simulink model "kinovaMicoSimscapeModel"  (R2021b)
(part 28 of 50)

Y4_10_2=(111*dq5*dqr3*sin(q4))/4000 - (111*dq5*dqr2*sin(q4))/4000 - dq5*dqr4*sin(q5)*((111*3^(1/2))/8000 + 1923/80000) + (111*dq5*dqr2*cos(2*q5)*sin(q4))/4000 + (111*dq5*dqr2*sin(2*q5)*cos(q4))/8000 - (111*dq5*dqr3*cos(2*q5)*sin(q4))/4000 - (111*dq5*dqr3*sin(2*q5)*cos(q4))/8000 + dq2*dqr2*sin(2*q4)*((37*3^(1/2))/16000 + 1923/80000) - dq2*dqr3*sin(2*q4)*((37*3^(1/2))/16000 + 1923/80000) - dq3*dqr2*sin(2*q4)*((37*3^(1/2))/16000 + 1923/80000) + dq3*dqr3*sin(2*q4)*((37*3^(1/2))/16000 + 1923/80000) - dq1*dqr1*sin(2*q4)*((37*3^(1/2))/32000 + 1923/160000) - (111*3^(1/2)*dq5*dqr4*sin(2*q5))/8000 - (29*3^(1/2)*dq1*dqr2*cos(q2)*sin(q4))/400 + (29*3^(1/2)*dq2*dqr2*cos(q4)*sin(q3))/400 - dq2*dqr2*cos(2*q4)*sin(q5)*((111*3^(1/2))/4000 + 1923/40000) + dq2*dqr3*cos(2*q4)*sin(q5)*((111*3^(1/2))/4000 + 1923/40000) + dq3*dqr2*cos(2*q4)*sin(q5)*((111*3^(1/2))/4000 + 1923/40000) - dq3*dqr3*cos(2*q4)*sin(q5)*((111*3^(1/2))/4000 + 1923/40000) - dq2*dqr2*sin(2*q4)*cos(q5)*((111*3^(1/2))/8000 + 1923/80000) + dq2*dqr3*sin(2*q4)*cos(q5)*((111*3^(1/2))/8000 + 1923/80000) + dq3*dqr2*sin(2*q4)*cos(q5)*((111*3^(1/2))/8000 + 1923/80000) - dq3*dqr3*sin(2*q4)*cos(q5)*((111*3^(1/2))/8000 + 1923/80000) + (111*dq1*dqr5*cos(q3)*cos(q4)*sin(q2))/4000 - (37*3^(1/2)*dq1*dqr1*cos(2*q4)*sin(2*q5))/8000 - (37*3^(1/2)*dq1*dqr1*cos(2*q5)*sin(2*q4))/6400 + (37*3^(1/2)*dq2*dqr2*cos(2*q4)*sin(2*q5))/4000 + (37*3^(1/2)*dq2*dqr2*cos(2*q5)*sin(2*q4))/3200 - (37*3^(1/2)*dq2*dqr3*cos(2*q4)*sin(2*q5))/4000 - (37*3^(1/2)*dq2*dqr3*cos(2*q5)*sin(2*q4))/3200 - (37*3^(1/2)*dq3*dqr2*cos(2*q4)*sin(2*q5))/4000 - (37*3^(1/2)*dq3*dqr2*cos(2*q5)*sin(2*q4))/3200 + (37*3^(1/2)*dq3*dqr3*cos(2*q4)*sin(2*q5))/4000 + (37*3^(1/2)*dq3*dqr3*cos(2*q5)*sin(2*q4))/3200 - dq5*dqr2*cos(q4)*sin(q5)*((1923*3^(1/2))/80000 + 333/8000) + dq5*dqr3*cos(q4)*sin(q5)*((1923*3^(1/2))/80000 + 333/8000) - dq1*dqr2*cos(q2)*sin(q3)*((333*3^(1/2))/16000 + 1923/80000) + dq1*dqr2*cos(q3)*sin(q2)*((333*3^(1/2))/16000 + 1923/80000) + dq1*dqr3*cos(q2)*sin(q3)*((333*3^(1/2))/16000 + 1923/80000) - dq1*dqr3*cos(q3)*sin(q2)*((333*3^(1/2))/16000 + 1923/80000) - (111*dq1*dqr2*cos(2*q5)*sin(q2)*sin(q3)*sin(q4))/8000 - (111*dq1*dqr2*sin(2*q5)*cos(q4)*sin(q2)*sin(q3))/4000 + (111*dq1*dqr3*cos(2*q5)*sin(q2)*sin(q3)*sin(q4))/8000 + (111*dq1*dqr3*sin(2*q5)*cos(q4)*sin(q2)*sin(q3))/4000 - (111*dq1*dqr5*sin(2*q5)*cos(q2)*sin(q3)*sin(q4))/8000 + (111*dq1*dqr5*sin(2*q5)*cos(q3)*sin(q2)*sin(q4))/8000 + (29*3^(1/2)*dq1*dqr2*cos(q2)*cos(q4)*sin(q5))/200 + (29*3^(1/2)*dq1*dqr2*cos(q2)*cos(q5)*sin(q4))/400 - (29*3^(1/2)*dq2*dqr2*cos(q4)*cos(q5)*sin(q3))/400 + dq1*dqr2*cos(2*q4)*cos(q2)*sin(q3)*((37*3^(1/2))/16000 + 1923/80000) - dq1*dqr2*cos(2*q4)*cos(q3)*sin(q2)*((37*3^(1/2))/16000 + 1923/80000) - dq1*dqr3*cos(2*q4)*cos(q2)*sin(q3)*((37*3^(1/2))/16000 + 1923/80000) + dq1*dqr3*cos(2*q4)*cos(q3)*sin(q2)*((37*3^(1/2))/16000 + 1923/80000) + (29*3^(1/2)*dq2*dqr2*sin(q3)*sin(q4)*sin(q5))/200 + (111*3^(1/2)*dq1*dqr2*cos(2*q5)*cos(q2)*sin(q3))/16000 - (111*3^(1/2)*dq1*dqr2*cos(2*q5)*cos(q3)*sin(q2))/16000 - (111*3^(1/2)*dq1*dqr3*cos(2*q5)*cos(q2)*sin(q3))/16000 + (111*3^(1/2)*dq1*dqr3*cos(2*q5)*cos(q3)*sin(q2))/16000 - (111*3^(1/2)*dq1*dqr5*sin(2*q5)*sin(q2)*sin(q3))/8000 + dq1*dqr2*cos(q2)*cos(q3)*sin(q4)*((2513*3^(1/2))/40000 - 37/8000) - dq1*dqr3*cos(q2)*cos(q3)*sin(q4)*((2513*3^(1/2))/40000 - 37/8000) + dq1*dqr2*cos(q2)*cos(q5)*sin(q3)*((111*3^(1/2))/8000 + 1923/80000) - dq1*dqr2*cos(q3)*cos(q5)*sin(q2)*((111*3^(1/2))/8000 + 1923/80000) - dq1*dqr3*cos(q2)*cos(q5)*sin(q3)*((111*3^(1/2))/8000 + 1923/80000) + dq1*dqr3*cos(q3)*cos(q5)*sin(q2)*((111*3^(1/2))/8000 + 1923/80000) - (111*dq1*dqr2*cos(2*q5)*cos(q2)*cos(q3)*sin(q4))/8000 - (111*dq1*dqr2*sin(2*q5)*cos(q2)*cos(q3)*cos(q4))/4000 + (111*dq1*dqr3*cos(2*q5)*cos(q2)*cos(q3)*sin(q4))/8000 + (111*dq1*dqr3*sin(2*q5)*cos(q2)*cos(q3)*cos(q4))/4000 - (111*dq1*dqr5*cos(2*q5)*cos(q3)*cos(q4)*sin(q2))/4000 + dq1*dqr2*sin(q2)*sin(q3)*sin(q4)*((2513*3^(1/2))/40000 - 37/8000) - dq1*dqr3*sin(q2)*sin(q3)*sin(q4)*((2513*3^(1/2))/40000 - 37/8000) - dq1*dqr5*sin(q2)*sin(q3)*sin(q5)*((111*3^(1/2))/8000 + 1923/80000) - dq1*dqr2*cos(2*q4)*cos(q2)*cos(q5)*sin(q3)*((111*3^(1/2))/8000 + 1923/80000) + dq1*dqr2*cos(2*q4)*cos(q3)*cos(q5)*sin(q2)*((111*3^(1/2))/8000 + 1923/80000) + dq1*dqr3*cos(2*q4)*cos(q2)*cos(q5)*sin(q3)*((111*3^(1/2))/8000 + 1923/80000) - dq1*dqr3*cos(2*q4)*cos(q3)*cos(q5)*sin(q2)*((111*3^(1/2))/8000 + 1923/80000) + dq1*dqr2*sin(2*q4)*cos(q2)*sin(q3)*sin(q5)*((111*3^(1/2))/4000 + 1923/40000) - dq1*dqr2*sin(2*q4)*cos(q3)*sin(q2)*sin(q5)*((111*3^(1/2))/4000 + 1923/40000) - dq1*dqr3*sin(2*q4)*cos(q2)*sin(q3)*sin(q5)*((111*3^(1/2))/4000 + 1923/40000) + dq1*dqr3*sin(2*q4)*cos(q3)*sin(q2)*sin(q5)*((111*3^(1/2))/4000 + 1923/40000) + (37*3^(1/2)*dq1*dqr1*cos(2*q2)*cos(2*q3)*cos(2*q4)*sin(2*q5))/8000 + (37*3^(1/2)*dq1*dqr2*cos(2*q4)*cos(2*q5)*cos(q2)*sin(q3))/3200 - (37*3^(1/2)*dq1*dqr2*cos(2*q4)*cos(2*q5)*cos(q3)*sin(q2))/3200 - (37*3^(1/2)*dq1*dqr3*cos(2*q4)*cos(2*q5)*cos(q2)*sin(q3))/3200 + (37*3^(1/2)*dq1*dqr3*cos(2*q4)*cos(2*q5)*cos(q3)*sin(q2))/3200 - dq1*dqr2*cos(q2)*cos(q3)*cos(q4)*sin(q5)*((877*3^(1/2))/8000 + 37/4000) + dq1*dqr3*cos(q2)*cos(q3)*cos(q4)*sin(q5)*((877*3^(1/2))/8000 + 37/4000) - dq1*dqr2*cos(q2)*cos(q3)*cos(q5)*sin(q4)*((1231*3^(1/2))/40000 - 37/1000) + dq1*dqr3*cos(q2)*cos(q3)*cos(q5)*sin(q4)*((1231*3^(1/2))/40000 - 37/1000) - (37*3^(1/2)*dq1*dqr2*sin(2*q4)*sin(2*q5)*cos(q2)*sin(q3))/4000 + (37*3^(1/2)*dq1*dqr2*sin(2*q4)*sin(2*q5)*cos(q3)*sin(q2))/4000 + (37*3^(1/2)*dq1*dqr3*sin(2*q4)*sin(2*q5)*cos(q2)*sin(q3))/4000 - (37*3^(1/2)*dq1*dqr3*sin(2*q4)*sin(2*q5)*cos(q3)*sin(q2))/4000 - dq1*dqr2*cos(q4)*sin(q2)*sin(q3)*sin(q5)*((877*3^(1/2))/8000 + 37/4000) + dq1*dqr3*cos(q4)*sin(q2)*sin(q3)*sin(q5)*((877*3^(1/2))/8000 + 37/4000) - dq1*dqr2*cos(q5)*sin(q2)*sin(q3)*sin(q4)*((1231*3^(1/2))/40000 - 37/1000) + dq1*dqr3*cos(q5)*sin(q2)*sin(q3)*sin(q4)*((1231*3^(1/2))/40000 - 37/1000) + dq1*dqr5*cos(q2)*sin(q3)*sin(q4)*sin(q5)*((1923*3^(1/2))/80000 + 333/8000) - dq1*dqr5*cos(q3)*sin(q2)*sin(q4)*sin(q5)*((1923*3^(1/2))/80000 + 333/8000);
Y4_10_3=(333*ddqr1*cos(q2 - q3 + q4 + 2*q5))/32000 - (111*ddqr1*cos(q2 - q3 + q4 - 2*q5))/32000 - (333*ddqr1*cos(q3 - q2 + q4 + 2*q5))/32000 - (37*3^(1/2)*ddqr5)/2000 + (111*ddqr1*cos(q2 - q3 - q4 + 2*q5))/32000 + (111*ddqr2*cos(q4 - 2*q5))/16000 - (333*ddqr2*cos(q4 + 2*q5))/16000 - (111*ddqr3*cos(q4 - 2*q5))/16000 + (333*ddqr3*cos(q4 + 2*q5))/16000 - ddqr4*((333*3^(1/2))/8000 + 1923/40000) - (111*dq2*dqr5*sin(q4))/4000 + (111*dq3*dqr5*sin(q4))/4000 - (29*3^(1/2)*ddqr1*cos(q2 - q4))/800 - (29*3^(1/2)*ddqr2*cos(q3 - q4))/800 + ddqr1*cos(q2 - q3 - q4 + q5)*((403*3^(1/2))/20000 + 37/3200) - ddqr1*cos(q2 - q3 + q4 - q5)*((771*3^(1/2))/40000 + 37/3200) - (87*3^(1/2)*ddqr1*cos(q2 + q4 + q5))/1600 + (87*3^(1/2)*ddqr2*cos(q3 + q4 + q5))/1600 + (111*3^(1/2)*ddqr4*cos(2*q5))/8000 + ddqr1*cos(q2 - q3 + q5)*((111*3^(1/2))/8000 + 1923/80000) + ddqr1*cos(q3 - q2 + q5)*((111*3^(1/2))/8000 + 1923/80000) - ddqr1*cos(q2 - q3 + q4)*((2443*3^(1/2))/80000 - 37/16000) + ddqr1*cos(q3 - q2 + q4)*((2583*3^(1/2))/80000 - 37/16000) - ddqr2*cos(q4 + q5)*((351*3^(1/2))/5000 - 111/8000) + ddqr3*cos(q4 + q5)*((351*3^(1/2))/5000 - 111/8000) + (29*3^(1/2)*ddqr1*cos(q2 + q4 - q5))/1600 - (29*3^(1/2)*ddqr1*cos(q2 - q4 + q5))/1600 + (87*3^(1/2)*ddqr1*cos(q4 - q2 + q5))/1600 - (29*3^(1/2)*ddqr2*cos(q3 + q4 - q5))/1600 - (29*3^(1/2)*ddqr2*cos(q3 - q4 + q5))/1600 + (87*3^(1/2)*ddqr2*cos(q4 - q3 + q5))/1600 + ddqr4*cos(q5)*((111*3^(1/2))/4000 + 1923/40000) + ddqr5*cos(q5)*((111*3^(1/2))/4000 + 1923/40000) + ddqr2*cos(q4)*((2513*3^(1/2))/40000 - 37/8000) - ddqr3*cos(q4)*((2513*3^(1/2))/40000 - 37/8000) + (29*3^(1/2)*ddqr1*cos(q2 + q4))/800 - (29*3^(1/2)*ddqr2*cos(q3 + q4))/800 + ddqr1*cos(q2 - q3 + q4 + q5)*((2703*3^(1/2))/80000 - 111/16000) - ddqr1*cos(q3 - q2 + q4 + q5)*((2913*3^(1/2))/80000 - 111/16000) + ddqr2*cos(q4 - q5)*((1577*3^(1/2))/40000 + 37/1600) - ddqr3*cos(q4 - q5)*((1577*3^(1/2))/40000 + 37/1600) - ddqr1*cos(q2 - q3)*((333*3^(1/2))/8000 + 1923/40000) + (111*3^(1/2)*ddqr1*cos(q2 - q3 + 2*q5))/16000 + (111*3^(1/2)*ddqr1*cos(q3 - q2 + 2*q5))/16000 - dq5*dqr5*sin(q5)*((111*3^(1/2))/4000 + 1923/40000) - dq4*dqr5*sin(q5)*((111*3^(1/2))/8000 + 1923/80000) + (111*dq2*dqr5*cos(2*q5)*sin(q4))/4000 + (111*dq2*dqr5*sin(2*q5)*cos(q4))/8000 - (111*dq3*dqr5*cos(2*q5)*sin(q4))/4000 - (111*dq3*dqr5*sin(2*q5)*cos(q4))/8000 - (111*3^(1/2)*dq4*dqr5*sin(2*q5))/8000 - (111*dq1*dqr5*cos(q2)*cos(q4)*sin(q3))/4000 - dq2*dqr5*cos(q4)*sin(q5)*((1923*3^(1/2))/80000 + 333/8000) + dq3*dqr5*cos(q4)*sin(q5)*((1923*3^(1/2))/80000 + 333/8000) - (111*3^(1/2)*dq1*dqr5*sin(2*q5)*cos(q2)*cos(q3))/8000 - dq1*dqr5*cos(q2)*cos(q3)*sin(q5)*((111*3^(1/2))/8000 + 1923/80000) + (111*dq1*dqr5*cos(2*q5)*cos(q2)*cos(q4)*sin(q3))/4000;
Y4_13_1=(37*sin(q2 - q3)*cos(q4))/1000;
Y4_14_1=(37*cos(q4 - q5)*sin(q2 - q3))/4000 - (111*sin(q2 - q3)*cos(q4 + q5))/4000 + sin(q2 - q3)*cos(q4)*((641*3^(1/2))/20000 + 37/1000);
Y4_18_1=(3*ddqr4)/4 + (3*ddqr1*cos(q2 - q3))/4 + (3*dq1*dqr1*sin(2*q4))/16 - (3*dq2*dqr2*sin(2*q4))/8 + (3*dq2*dqr3*sin(2*q4))/8 + (3*dq3*dqr2*sin(2*q4))/8 - (3*dq3*dqr3*sin(2*q4))/8 + (3^(1/2)*ddqr1*cos(q2 - q3 + q4))/8 - (3^(1/2)*ddqr1*cos(q3 - q2 + q4))/8 - (3^(1/2)*ddqr2*cos(q4))/4 + (3^(1/2)*ddqr3*cos(q4))/4 + (3*dq1*dqr2*cos(q2)*sin(q3))/8 - (3*dq1*dqr2*cos(q3)*sin(q2))/8 + (3*dq2*dqr1*cos(q2)*sin(q3))/8 - (3*dq2*dqr1*cos(q3)*sin(q2))/8 - (3*dq1*dqr3*cos(q2)*sin(q3))/8 + (3*dq1*dqr3*cos(q3)*sin(q2))/8 - (3*dq3*dqr1*cos(q2)*sin(q3))/8 + (3*dq3*dqr1*cos(q3)*sin(q2))/8 - (3*dq1*dqr2*cos(2*q4)*cos(q2)*sin(q3))/8 + (3*dq1*dqr2*cos(2*q4)*cos(q3)*sin(q2))/8 - (3*dq2*dqr1*cos(2*q4)*cos(q2)*sin(q3))/8 + (3*dq2*dqr1*cos(2*q4)*cos(q3)*sin(q2))/8 + (3*dq1*dqr3*cos(2*q4)*cos(q2)*sin(q3))/8 - (3*dq1*dqr3*cos(2*q4)*cos(q3)*sin(q2))/8 + (3*dq3*dqr1*cos(2*q4)*cos(q2)*sin(q3))/8 - (3*dq3*dqr1*cos(2*q4)*cos(q3)*sin(q2))/8 - (3*dq1*dqr1*cos(2*q2)*cos(2*q3)*sin(2*q4))/16 - (3*dq1*dqr1*sin(2*q2)*sin(2*q3)*sin(2*q4))/16 - (3^(1/2)*dq1*dqr2*cos(q2)*cos(q3)*sin(q4))/4 - (3^(1/2)*dq2*dqr1*cos(q2)*cos(q3)*sin(q4))/4 + (3^(1/2)*dq1*dqr3*cos(q2)*cos(q3)*sin(q4))/4 + (3^(1/2)*dq3*dqr1*cos(q2)*cos(q3)*sin(q4))/4 - (3^(1/2)*dq1*dqr2*sin(q2)*sin(q3)*sin(q4))/4 - (3^(1/2)*dq2*dqr1*sin(q2)*sin(q3)*sin(q4))/4 + (3^(1/2)*dq1*dqr3*sin(q2)*sin(q3)*sin(q4))/4 + (3^(1/2)*dq3*dqr1*sin(q2)*sin(q3)*sin(q4))/4 - (3^(1/2)*dq1*dqr1*cos(2*q2)*sin(2*q3)*cos(q4))/8 + (3^(1/2)*dq1*dqr1*cos(2*q3)*sin(2*q2)*cos(q4))/8;
Y4_19_1=(3*dq1*dqr1*cos(2*q4)*sin(2*q5))/32 - (3*dq1*dqr1*cos(2*q4)*sin(q5))/16 - (3*dq1*dqr1*sin(2*q4)*cos(q5))/32 - (3*dq1*dqr1*sin(2*q4))/128 + (15*dq1*dqr1*cos(2*q5)*sin(2*q4))/128 + (21*dq2*dqr1*cos(q2)*sin(q3))/64 - (21*dq2*dqr1*cos(q3)*sin(q2))/64 - (21*dq3*dqr1*cos(q2)*sin(q3))/64 + (21*dq3*dqr1*cos(q3)*sin(q2))/64 - (3*dq1*dqr2*cos(2*q4)*cos(q3)*sin(q2))/64 + (3*dq2*dqr1*cos(2*q4)*cos(q2)*sin(q3))/64 - (3*dq2*dqr1*cos(2*q4)*cos(q3)*sin(q2))/64 - (9*dq2*dqr1*cos(2*q5)*cos(q2)*sin(q3))/64 + (9*dq2*dqr1*cos(2*q5)*cos(q3)*sin(q2))/64 - (3*dq3*dqr1*cos(2*q4)*cos(q2)*sin(q3))/64 + (3*dq3*dqr1*cos(2*q4)*cos(q3)*sin(q2))/64 + (9*dq3*dqr1*cos(2*q5)*cos(q2)*sin(q3))/64 - (9*dq3*dqr1*cos(2*q5)*cos(q3)*sin(q2))/64 + (9*dq5*dqr1*sin(2*q5)*cos(q2)*cos(q3))/32 + (9*dq5*dqr1*sin(2*q5)*sin(q2)*sin(q3))/32 + (3*dq1*dqr2*cos(q3)*cos(q5)*sin(q2))/16 - (3*dq2*dqr1*cos(q2)*cos(q5)*sin(q3))/16 + (3*dq2*dqr1*cos(q3)*cos(q5)*sin(q2))/16 + (3*dq3*dqr1*cos(q2)*cos(q5)*sin(q3))/16 - (3*dq3*dqr1*cos(q3)*cos(q5)*sin(q2))/16 + (3*dq5*dqr1*cos(q2)*cos(q3)*sin(q5))/16 + (3*dq1*dqr1*cos(2*q2)*cos(2*q3)*sin(2*q4))/128 + (3*dq5*dqr1*sin(q2)*sin(q3)*sin(q5))/16 + (3*dq1*dqr1*sin(2*q2)*sin(2*q3)*sin(2*q4))/128 - (3*dq1*dqr1*cos(2*q2)*cos(2*q3)*cos(2*q4)*sin(2*q5))/32 - (15*dq1*dqr1*cos(2*q2)*cos(2*q3)*cos(2*q5)*sin(2*q4))/128 + (3*dq1*dqr2*sin(2*q4)*cos(q3)*sin(q2)*sin(q5))/8 - (3*dq2*dqr1*sin(2*q4)*cos(q2)*sin(q3)*sin(q5))/8 + (3*dq2*dqr1*sin(2*q4)*cos(q3)*sin(q2)*sin(q5))/8 + (3*dq3*dqr1*sin(2*q4)*cos(q2)*sin(q3)*sin(q5))/8 - (3*dq3*dqr1*sin(2*q4)*cos(q3)*sin(q2)*sin(q5))/8 + (3^(1/2)*dq2*dqr1*cos(q2)*cos(q3)*sin(q4))/32 - (3^(1/2)*dq3*dqr1*cos(q2)*cos(q3)*sin(q4))/32 + (3*3^(1/2)*dq5*dqr1*cos(q2)*cos(q4)*sin(q3))/16 - (3*3^(1/2)*dq5*dqr1*cos(q3)*cos(q4)*sin(q2))/16 - (3*dq1*dqr1*cos(2*q4)*sin(2*q2)*sin(2*q3)*sin(2*q5))/32 - (15*dq1*dqr1*cos(2*q5)*sin(2*q2)*sin(2*q3)*sin(2*q4))/128 + (3^(1/2)*dq1*dqr2*sin(q2)*sin(q3)*sin(q4))/32 + (3^(1/2)*dq2*dqr1*sin(q2)*sin(q3)*sin(q4))/32 - (3^(1/2)*dq3*dqr1*sin(q2)*sin(q3)*sin(q4))/32 + (15*dq1*dqr2*cos(2*q4)*cos(2*q5)*cos(q3)*sin(q2))/64 - (15*dq2*dqr1*cos(2*q4)*cos(2*q5)*cos(q2)*sin(q3))/64 + (15*dq2*dqr1*cos(2*q4)*cos(2*q5)*cos(q3)*sin(q2))/64 + (15*dq3*dqr1*cos(2*q4)*cos(2*q5)*cos(q2)*sin(q3))/64 - (15*dq3*dqr1*cos(2*q4)*cos(2*q5)*cos(q3)*sin(q2))/64 - (3*dq1*dqr2*sin(2*q4)*sin(2*q5)*cos(q3)*sin(q2))/16 + (3*dq2*dqr1*sin(2*q4)*sin(2*q5)*cos(q2)*sin(q3))/16 - (3*dq2*dqr1*sin(2*q4)*sin(2*q5)*cos(q3)*sin(q2))/16 - (3*dq3*dqr1*sin(2*q4)*sin(2*q5)*cos(q2)*sin(q3))/16 + (3*dq3*dqr1*sin(2*q4)*sin(2*q5)*cos(q3)*sin(q2))/16 + (3*dq1*dqr1*cos(2*q2)*cos(2*q3)*cos(2*q4)*sin(q5))/16 + (3*dq1*dqr1*cos(2*q2)*cos(2*q3)*sin(2*q4)*cos(q5))/32 + (3*dq1*dqr1*cos(2*q4)*sin(2*q2)*sin(2*q3)*sin(q5))/16 + (3*dq1*dqr1*sin(2*q2)*sin(2*q3)*sin(2*q4)*cos(q5))/32 + (3^(1/2)*dq1*dqr1*cos(2*q2)*sin(2*q3)*cos(q4))/64 - (3^(1/2)*dq1*dqr1*cos(2*q3)*sin(2*q2)*cos(q4))/64 - (3*dq1*dqr2*cos(2*q4)*cos(q3)*cos(q5)*sin(q2))/16 + (3*dq2*dqr1*cos(2*q4)*cos(q2)*cos(q5)*sin(q3))/16 - (3*dq2*dqr1*cos(2*q4)*cos(q3)*cos(q5)*sin(q2))/16 - (3*dq3*dqr1*cos(2*q4)*cos(q2)*cos(q5)*sin(q3))/16 + (3*dq3*dqr1*cos(2*q4)*cos(q3)*cos(q5)*sin(q2))/16 + (3*3^(1/2)*dq1*dqr1*cos(2*q2)*cos(2*q5)*sin(2*q3)*cos(q4))/64 - (3*3^(1/2)*dq1*dqr1*cos(2*q3)*cos(2*q5)*sin(2*q2)*cos(q4))/64 + (3^(1/2)*dq1*dqr2*cos(q4)*sin(q2)*sin(q3)*sin(q5))/8 - (3^(1/2)*dq1*dqr2*cos(q5)*sin(q2)*sin(q3)*sin(q4))/8 + (3^(1/2)*dq2*dqr1*cos(q4)*sin(q2)*sin(q3)*sin(q5))/8 - (3^(1/2)*dq2*dqr1*cos(q5)*sin(q2)*sin(q3)*sin(q4))/8 - (3^(1/2)*dq3*dqr1*cos(q4)*sin(q2)*sin(q3)*sin(q5))/8 + (3^(1/2)*dq3*dqr1*cos(q5)*sin(q2)*sin(q3)*sin(q4))/8 - (3*3^(1/2)*dq5*dqr1*cos(q2)*sin(q3)*sin(q4)*sin(q5))/16 + (3*3^(1/2)*dq5*dqr1*cos(q3)*sin(q2)*sin(q4)*sin(q5))/16 - (3*3^(1/2)*dq1*dqr1*cos(2*q2)*sin(2*q3)*sin(2*q5)*sin(q4))/32 + (3*3^(1/2)*dq1*dqr1*cos(2*q3)*sin(2*q2)*sin(2*q5)*sin(q4))/32 + (3*3^(1/2)*dq2*dqr1*cos(2*q5)*cos(q2)*cos(q3)*sin(q4))/32 + (3*3^(1/2)*dq2*dqr1*sin(2*q5)*cos(q2)*cos(q3)*cos(q4))/16 - (3*3^(1/2)*dq3*dqr1*cos(2*q5)*cos(q2)*cos(q3)*sin(q4))/32 - (3*3^(1/2)*dq3*dqr1*sin(2*q5)*cos(q2)*cos(q3)*cos(q4))/16 - (3*3^(1/2)*dq5*dqr1*cos(2*q5)*cos(q2)*cos(q4)*sin(q3))/16 + (3*3^(1/2)*dq5*dqr1*cos(2*q5)*cos(q3)*cos(q4)*sin(q2))/16 + (3*3^(1/2)*dq1*dqr2*cos(2*q5)*sin(q2)*sin(q3)*sin(q4))/32 + (3*3^(1/2)*dq1*dqr2*sin(2*q5)*cos(q4)*sin(q2)*sin(q3))/16 + (3*3^(1/2)*dq2*dqr1*cos(2*q5)*sin(q2)*sin(q3)*sin(q4))/32 + (3*3^(1/2)*dq2*dqr1*sin(2*q5)*cos(q4)*sin(q2)*sin(q3))/16 - (3*3^(1/2)*dq3*dqr1*cos(2*q5)*sin(q2)*sin(q3)*sin(q4))/32 - (3*3^(1/2)*dq3*dqr1*sin(2*q5)*cos(q4)*sin(q2)*sin(q3))/16 + (3*3^(1/2)*dq5*dqr1*sin(2*q5)*cos(q2)*sin(q3)*sin(q4))/32 - (3*3^(1/2)*dq5*dqr1*sin(2*q5)*cos(q3)*sin(q2)*sin(q4))/32 - (3^(1/2)*dq1*dqr1*cos(2*q2)*sin(2*q3)*cos(q4)*cos(q5))/16 + (3^(1/2)*dq1*dqr1*cos(2*q3)*sin(2*q2)*cos(q4)*cos(q5))/16 - (3^(1/2)*dq1*dqr1*cos(2*q2)*sin(2*q3)*sin(q4)*sin(q5))/16 + (3^(1/2)*dq1*dqr1*cos(2*q3)*sin(2*q2)*sin(q4)*sin(q5))/16 + (3^(1/2)*dq2*dqr1*cos(q2)*cos(q3)*cos(q4)*sin(q5))/8 - (3^(1/2)*dq2*dqr1*cos(q2)*cos(q3)*cos(q5)*sin(q4))/8 - (3^(1/2)*dq3*dqr1*cos(q2)*cos(q3)*cos(q4)*sin(q5))/8 + (3^(1/2)*dq3*dqr1*cos(q2)*cos(q3)*cos(q5)*sin(q4))/8;
Y4_19_2=(21*ddqr1*cos(q2 - q3))/32 - (9*ddqr1*cos(q3 - q2 + 2*q5))/64 - (9*ddqr1*cos(q2 - q3 + 2*q5))/64 + (3*dq4*dqr5*sin(q5))/16 + (3*dq5*dqr4*sin(q5))/16 + (3*dq5*dqr5*sin(q5))/8 + (3^(1/2)*ddqr1*cos(q2 - q3 + q4 - q5))/16 - (3^(1/2)*ddqr1*cos(q2 - q3 - q4 + q5))/16 + (3*dq2*dqr2*sin(2*q4))/64 - (3*dq2*dqr3*sin(2*q4))/64 - (3*dq3*dqr2*sin(2*q4))/64 + (3*dq3*dqr3*sin(2*q4))/64 + (9*dq4*dqr5*sin(2*q5))/32 + (9*dq5*dqr4*sin(2*q5))/32 - (3*3^(1/2)*ddqr1*cos(q2 - q3 - q4 + 2*q5))/128 + (3*dq2*dqr2*cos(2*q4)*sin(q5))/8 + (3*dq2*dqr2*sin(2*q4)*cos(q5))/16 - (3*dq2*dqr3*cos(2*q4)*sin(q5))/8 - (3*dq2*dqr3*sin(2*q4)*cos(q5))/16 - (3*dq3*dqr2*cos(2*q4)*sin(q5))/8 - (3*dq3*dqr2*sin(2*q4)*cos(q5))/16 + (3*dq3*dqr3*cos(2*q4)*sin(q5))/8 + (3*dq3*dqr3*sin(2*q4)*cos(q5))/16 + (3*3^(1/2)*dq2*dqr5*sin(q4))/16 + (3*3^(1/2)*dq5*dqr2*sin(q4))/16 - (3*3^(1/2)*dq3*dqr5*sin(q4))/16 - (3*3^(1/2)*dq5*dqr3*sin(q4))/16 - (3*dq2*dqr2*cos(2*q4)*sin(2*q5))/16 - (15*dq2*dqr2*cos(2*q5)*sin(2*q4))/64 + (3*dq2*dqr3*cos(2*q4)*sin(2*q5))/16 + (15*dq2*dqr3*cos(2*q5)*sin(2*q4))/64 + (3*dq3*dqr2*cos(2*q4)*sin(2*q5))/16 + (15*dq3*dqr2*cos(2*q5)*sin(2*q4))/64 - (3*dq3*dqr3*cos(2*q4)*sin(2*q5))/16 - (15*dq3*dqr3*cos(2*q5)*sin(2*q4))/64 + (21*dq1*dqr2*cos(q2)*sin(q3))/64 - (21*dq1*dqr2*cos(q3)*sin(q2))/64 - (21*dq1*dqr3*cos(q2)*sin(q3))/64 + (21*dq1*dqr3*cos(q3)*sin(q2))/64 + (3*dq1*dqr2*cos(2*q4)*cos(q2)*sin(q3))/64 - (9*dq1*dqr2*cos(2*q5)*cos(q2)*sin(q3))/64 + (9*dq1*dqr2*cos(2*q5)*cos(q3)*sin(q2))/64 - (3*dq1*dqr3*cos(2*q4)*cos(q2)*sin(q3))/64 + (3*dq1*dqr3*cos(2*q4)*cos(q3)*sin(q2))/64 + (9*dq1*dqr3*cos(2*q5)*cos(q2)*sin(q3))/64 - (9*dq1*dqr3*cos(2*q5)*cos(q3)*sin(q2))/64 + (9*dq1*dqr5*sin(2*q5)*cos(q2)*cos(q3))/32 + (9*dq1*dqr5*sin(2*q5)*sin(q2)*sin(q3))/32 + (3*3^(1/2)*dq2*dqr5*cos(q4)*sin(q5))/16 + (3*3^(1/2)*dq5*dqr2*cos(q4)*sin(q5))/16 - (3*3^(1/2)*dq3*dqr5*cos(q4)*sin(q5))/16 - (3*3^(1/2)*dq5*dqr3*cos(q4)*sin(q5))/16 - (3*3^(1/2)*dq2*dqr5*cos(2*q5)*sin(q4))/16 - (3*3^(1/2)*dq2*dqr5*sin(2*q5)*cos(q4))/32 - (3*3^(1/2)*dq5*dqr2*cos(2*q5)*sin(q4))/16 - (3*3^(1/2)*dq5*dqr2*sin(2*q5)*cos(q4))/32 + (3*3^(1/2)*dq3*dqr5*cos(2*q5)*sin(q4))/16 + (3*3^(1/2)*dq3*dqr5*sin(2*q5)*cos(q4))/32 + (3*3^(1/2)*dq5*dqr3*cos(2*q5)*sin(q4))/16 + (3*3^(1/2)*dq5*dqr3*sin(2*q5)*cos(q4))/32 - (3*dq1*dqr2*cos(q2)*cos(q5)*sin(q3))/16 + (3*dq1*dqr3*cos(q2)*cos(q5)*sin(q3))/16 - (3*dq1*dqr3*cos(q3)*cos(q5)*sin(q2))/16 + (3*dq1*dqr5*cos(q2)*cos(q3)*sin(q5))/16 + (3*dq1*dqr5*sin(q2)*sin(q3)*sin(q5))/16 - (3*dq1*dqr2*sin(2*q4)*cos(q2)*sin(q3)*sin(q5))/8 + (3*dq1*dqr3*sin(2*q4)*cos(q2)*sin(q3)*sin(q5))/8 - (3*dq1*dqr3*sin(2*q4)*cos(q3)*sin(q2)*sin(q5))/8 + (3^(1/2)*dq1*dqr2*cos(q2)*cos(q3)*sin(q4))/32 - (3^(1/2)*dq1*dqr3*cos(q2)*cos(q3)*sin(q4))/32 + (3*3^(1/2)*dq1*dqr5*cos(q2)*cos(q4)*sin(q3))/16 - (3*3^(1/2)*dq1*dqr5*cos(q3)*cos(q4)*sin(q2))/16 - (3^(1/2)*dq1*dqr3*sin(q2)*sin(q3)*sin(q4))/32 - (15*dq1*dqr2*cos(2*q4)*cos(2*q5)*cos(q2)*sin(q3))/64 + (15*dq1*dqr3*cos(2*q4)*cos(2*q5)*cos(q2)*sin(q3))/64 - (15*dq1*dqr3*cos(2*q4)*cos(2*q5)*cos(q3)*sin(q2))/64 + (3*dq1*dqr2*sin(2*q4)*sin(2*q5)*cos(q2)*sin(q3))/16 - (3*dq1*dqr3*sin(2*q4)*sin(2*q5)*cos(q2)*sin(q3))/16 + (3*dq1*dqr3*sin(2*q4)*sin(2*q5)*cos(q3)*sin(q2))/16 + (3*dq1*dqr2*cos(2*q4)*cos(q2)*cos(q5)*sin(q3))/16 - (3*dq1*dqr3*cos(2*q4)*cos(q2)*cos(q5)*sin(q3))/16 + (3*dq1*dqr3*cos(2*q4)*cos(q3)*cos(q5)*sin(q2))/16 - (3^(1/2)*dq1*dqr3*cos(q4)*sin(q2)*sin(q3)*sin(q5))/8 + (3^(1/2)*dq1*dqr3*cos(q5)*sin(q2)*sin(q3)*sin(q4))/8 - (3*3^(1/2)*dq1*dqr5*cos(q2)*sin(q3)*sin(q4)*sin(q5))/16 + (3*3^(1/2)*dq1*dqr5*cos(q3)*sin(q2)*sin(q4)*sin(q5))/16 + (3*3^(1/2)*dq1*dqr2*cos(2*q5)*cos(q2)*cos(q3)*sin(q4))/32 + (3*3^(1/2)*dq1*dqr2*sin(2*q5)*cos(q2)*cos(q3)*cos(q4))/16 - (3*3^(1/2)*dq1*dqr3*cos(2*q5)*cos(q2)*cos(q3)*sin(q4))/32 - (3*3^(1/2)*dq1*dqr3*sin(2*q5)*cos(q2)*cos(q3)*cos(q4))/16 - (3*3^(1/2)*dq1*dqr5*cos(2*q5)*cos(q2)*cos(q4)*sin(q3))/16 + (3*3^(1/2)*dq1*dqr5*cos(2*q5)*cos(q3)*cos(q4)*sin(q2))/16 - (3*3^(1/2)*dq1*dqr3*cos(2*q5)*sin(q2)*sin(q3)*sin(q4))/32 - (3*3^(1/2)*dq1*dqr3*sin(2*q5)*cos(q4)*sin(q2)*sin(q3))/16 + (3*3^(1/2)*dq1*dqr5*sin(2*q5)*cos(q2)*sin(q3)*sin(q4))/32 - (3*3^(1/2)*dq1*dqr5*sin(2*q5)*cos(q3)*sin(q2)*sin(q4))/32 + (3^(1/2)*dq1*dqr2*cos(q2)*cos(q3)*cos(q4)*sin(q5))/8 - (3^(1/2)*dq1*dqr2*cos(q2)*cos(q3)*cos(q5)*sin(q4))/8 - (3^(1/2)*dq1*dqr3*cos(q2)*cos(q3)*cos(q4)*sin(q5))/8 + (3^(1/2)*dq1*dqr3*cos(q2)*cos(q3)*cos(q5)*sin(q4))/8;
Y4_19_3=(21*ddqr4)/32 + (3*ddqr5)/8 - (3*ddqr1*cos(q2 - q3 + q5))/16 - (3*ddqr1*cos(q3 - q2 + q5))/16 - (3*ddqr4*cos(q5))/8 - (3*ddqr5*cos(q5))/8 - (9*ddqr4*cos(2*q5))/32 - (3^(1/2)*ddqr2*cos(q4 - q5))/8 - (3*3^(1/2)*ddqr2*cos(q4 - 2*q5))/64 + (9*3^(1/2)*ddqr2*cos(q4 + 2*q5))/64 + (3^(1/2)*ddqr3*cos(q4 - q5))/8 + (3*3^(1/2)*ddqr3*cos(q4 - 2*q5))/64 - (9*3^(1/2)*ddqr3*cos(q4 + 2*q5))/64 + (3*3^(1/2)*ddqr1*cos(q2 - q3 + q4 - 2*q5))/128 - (9*3^(1/2)*ddqr1*cos(q2 - q3 + q4 + 2*q5))/128 + (9*3^(1/2)*ddqr1*cos(q3 - q2 + q4 + 2*q5))/128 - (3^(1/2)*ddqr1*cos(q2 - q3 + q4))/64 + (3^(1/2)*ddqr1*cos(q3 - q2 + q4))/64 + (3^(1/2)*ddqr2*cos(q4))/32 - (3^(1/2)*ddqr3*cos(q4))/32;
Y4_23_1=-(3^(1/2)*sin(q2 - q3)*cos(q4))/2;
Y4_24_1=(3*3^(1/2)*sin(q2 - q3)*cos(q4 + q5))/8 - (3^(1/2)*sin(q2 - q3)*cos(q4))/4 - (3^(1/2)*cos(q4 - q5)*sin(q2 - q3))/8;
Y5_5_1=dq1*dqr1*sin(q5)*((253339*3^(1/2))/160000000 - 4107/8000000) - (4107*dq1*dqr1*sin(2*q5))/32000000 + (1369*dq1*dqr1*cos(2*q4)*sin(2*q5))/6400000 + (1369*dq1*dqr1*cos(2*q5)*sin(2*q4))/8000000 + (1369*dq2*dqr1*cos(q2)*sin(q3))/4000000 - (1369*dq2*dqr1*cos(q3)*sin(q2))/4000000 - (1369*dq3*dqr1*cos(q2)*sin(q3))/4000000 + (1369*dq3*dqr1*cos(q3)*sin(q2))/4000000 + (259*dq1*dqr1*cos(q4)*sin(q5))/2000000 + (259*dq1*dqr1*cos(q5)*sin(q4))/1000000 - (4107*dq4*dqr1*sin(2*q5)*cos(q2)*cos(q3))/8000000 - (4107*dq4*dqr1*sin(2*q5)*sin(q2)*sin(q3))/8000000 - (1073*3^(1/2)*dq1*dqr1*cos(q3)*sin(q5))/400000 - dq1*dqr1*sin(2*q4)*cos(q5)*((23717*3^(1/2))/80000000 + 1369/4000000) - dq1*dqr1*cos(2*q4)*sin(q5)*((23717*3^(1/2))/160000000 + 1369/8000000) + (1073*dq1*dqr1*cos(q4)*cos(q5)*sin(q3))/200000 - (1073*dq2*dqr1*cos(q2)*cos(q4)*sin(q5))/200000 - (1073*dq2*dqr1*cos(q2)*cos(q5)*sin(q4))/100000 - (12321*dq1*dqr1*cos(2*q2)*cos(2*q3)*sin(2*q5))/32000000 - (1073*dq1*dqr1*sin(q3)*sin(q4)*sin(q5))/400000 - (12321*dq1*dqr1*sin(2*q2)*sin(2*q3)*sin(2*q5))/32000000 - (1369*dq1*dqr1*cos(2*q2)*cos(2*q3)*cos(2*q4)*sin(2*q5))/6400000 - (1369*dq1*dqr1*cos(2*q2)*cos(2*q3)*cos(2*q5)*sin(2*q4))/8000000 + (1073*dq1*dqr1*cos(2*q2)*sin(q3)*sin(q4)*sin(q5))/400000 - (1073*dq1*dqr1*sin(2*q2)*cos(q3)*sin(q4)*sin(q5))/400000 + (1369*3^(1/2)*dq2*dqr1*cos(q2)*cos(q3)*sin(q4))/4000000 - (1369*3^(1/2)*dq3*dqr1*cos(q2)*cos(q3)*sin(q4))/4000000 - (1369*3^(1/2)*dq4*dqr1*cos(q2)*cos(q4)*sin(q3))/4000000 + (1369*3^(1/2)*dq4*dqr1*cos(q3)*cos(q4)*sin(q2))/4000000 - (1369*dq1*dqr1*cos(2*q4)*sin(2*q2)*sin(2*q3)*sin(2*q5))/6400000 - (1369*dq1*dqr1*cos(2*q5)*sin(2*q2)*sin(2*q3)*sin(2*q4))/8000000 + (1369*3^(1/2)*dq1*dqr2*sin(q2)*sin(q3)*sin(q4))/4000000 + (1369*3^(1/2)*dq2*dqr1*sin(q2)*sin(q3)*sin(q4))/4000000 - (1369*3^(1/2)*dq3*dqr1*sin(q2)*sin(q3)*sin(q4))/4000000 + (32449*dq1*dqr1*cos(2*q2)*sin(2*q3)*cos(q4)*cos(q5))/8000000 - (32449*dq1*dqr1*cos(2*q3)*sin(2*q2)*cos(q4)*cos(q5))/8000000 - (1369*dq2*dqr1*cos(2*q4)*cos(2*q5)*cos(q2)*sin(q3))/4000000 + (1369*dq2*dqr1*cos(2*q4)*cos(2*q5)*cos(q3)*sin(q2))/4000000 + (1369*dq3*dqr1*cos(2*q4)*cos(2*q5)*cos(q2)*sin(q3))/4000000 - (1369*dq3*dqr1*cos(2*q4)*cos(2*q5)*cos(q3)*sin(q2))/4000000 + (1369*dq2*dqr1*sin(2*q4)*sin(2*q5)*cos(q2)*sin(q3))/3200000 - (1369*dq2*dqr1*sin(2*q4)*sin(2*q5)*cos(q3)*sin(q2))/3200000 - (1369*dq3*dqr1*sin(2*q4)*sin(2*q5)*cos(q2)*sin(q3))/3200000 + (1369*dq3*dqr1*sin(2*q4)*sin(2*q5)*cos(q3)*sin(q2))/3200000 + (1073*3^(1/2)*dq1*dqr1*cos(2*q2)*cos(q3)*sin(q5))/400000 + (32449*dq2*dqr1*cos(q2)*cos(q3)*cos(q4)*sin(q5))/8000000 + (32449*dq2*dqr1*cos(q2)*cos(q3)*cos(q5)*sin(q4))/4000000 - (32449*dq3*dqr1*cos(q2)*cos(q3)*cos(q4)*sin(q5))/8000000 - (32449*dq3*dqr1*cos(q2)*cos(q3)*cos(q5)*sin(q4))/4000000 + (1073*3^(1/2)*dq1*dqr1*sin(2*q2)*sin(q3)*sin(q5))/400000 - dq1*dqr1*cos(2*q2)*cos(2*q3)*sin(q5)*((348207*3^(1/2))/160000000 + 1369/8000000) + (32449*dq1*dqr2*cos(q4)*sin(q2)*sin(q3)*sin(q5))/8000000 + (32449*dq1*dqr2*cos(q5)*sin(q2)*sin(q3)*sin(q4))/4000000 + (32449*dq2*dqr1*cos(q4)*sin(q2)*sin(q3)*sin(q5))/8000000 + (32449*dq2*dqr1*cos(q5)*sin(q2)*sin(q3)*sin(q4))/4000000 - (32449*dq3*dqr1*cos(q4)*sin(q2)*sin(q3)*sin(q5))/8000000 - (32449*dq3*dqr1*cos(q5)*sin(q2)*sin(q3)*sin(q4))/4000000 - dq1*dqr1*sin(2*q2)*sin(2*q3)*sin(q5)*((348207*3^(1/2))/160000000 + 1369/8000000) - dq2*dqr1*cos(q2)*cos(q5)*sin(q3)*((23717*3^(1/2))/40000000 + 1369/2000000) + dq2*dqr1*cos(q3)*cos(q5)*sin(q2)*((23717*3^(1/2))/40000000 + 1369/2000000) + dq3*dqr1*cos(q2)*cos(q5)*sin(q3)*((23717*3^(1/2))/40000000 + 1369/2000000) - dq3*dqr1*cos(q3)*cos(q5)*sin(q2)*((23717*3^(1/2))/40000000 + 1369/2000000) - dq4*dqr1*cos(q2)*cos(q3)*sin(q5)*((23717*3^(1/2))/40000000 + 1369/2000000) - (1073*dq1*dqr1*cos(2*q2)*cos(q4)*cos(q5)*sin(q3))/200000 + (1073*dq1*dqr1*sin(2*q2)*cos(q3)*cos(q4)*cos(q5))/200000 - dq4*dqr1*sin(q2)*sin(q3)*sin(q5)*((23717*3^(1/2))/40000000 + 1369/2000000) + (1369*3^(1/2)*dq1*dqr1*cos(2*q2)*cos(2*q5)*sin(2*q3)*cos(q4))/4000000 - (1369*3^(1/2)*dq1*dqr1*cos(2*q3)*cos(2*q5)*sin(2*q2)*cos(q4))/4000000 + dq2*dqr1*cos(2*q4)*cos(q2)*cos(q5)*sin(q3)*((23717*3^(1/2))/40000000 + 1369/2000000) - dq2*dqr1*cos(2*q4)*cos(q3)*cos(q5)*sin(q2)*((23717*3^(1/2))/40000000 + 1369/2000000) - dq3*dqr1*cos(2*q4)*cos(q2)*cos(q5)*sin(q3)*((23717*3^(1/2))/40000000 + 1369/2000000) + dq3*dqr1*cos(2*q4)*cos(q3)*cos(q5)*sin(q2)*((23717*3^(1/2))/40000000 + 1369/2000000) - (1369*3^(1/2)*dq1*dqr1*cos(2*q2)*sin(2*q3)*sin(2*q5)*sin(q4))/8000000 + (1369*3^(1/2)*dq1*dqr1*cos(2*q3)*sin(2*q2)*sin(2*q5)*sin(q4))/8000000 - dq2*dqr1*sin(2*q4)*cos(q2)*sin(q3)*sin(q5)*((23717*3^(1/2))/80000000 + 1369/4000000) + dq2*dqr1*sin(2*q4)*cos(q3)*sin(q2)*sin(q5)*((23717*3^(1/2))/80000000 + 1369/4000000) + dq3*dqr1*sin(2*q4)*cos(q2)*sin(q3)*sin(q5)*((23717*3^(1/2))/80000000 + 1369/4000000) - dq3*dqr1*sin(2*q4)*cos(q3)*sin(q2)*sin(q5)*((23717*3^(1/2))/80000000 + 1369/4000000) + (1369*3^(1/2)*dq2*dqr1*cos(2*q5)*cos(q2)*cos(q3)*sin(q4))/4000000 + (1369*3^(1/2)*dq2*dqr1*sin(2*q5)*cos(q2)*cos(q3)*cos(q4))/8000000 - (1369*3^(1/2)*dq3*dqr1*cos(2*q5)*cos(q2)*cos(q3)*sin(q4))/4000000 - (1369*3^(1/2)*dq3*dqr1*sin(2*q5)*cos(q2)*cos(q3)*cos(q4))/8000000 + (1369*3^(1/2)*dq4*dqr1*cos(2*q5)*cos(q2)*cos(q4)*sin(q3))/4000000 - (1369*3^(1/2)*dq4*dqr1*cos(2*q5)*cos(q3)*cos(q4)*sin(q2))/4000000 + (1369*3^(1/2)*dq1*dqr2*cos(2*q5)*sin(q2)*sin(q3)*sin(q4))/4000000 + (1369*3^(1/2)*dq1*dqr2*sin(2*q5)*cos(q4)*sin(q2)*sin(q3))/8000000 + (1369*3^(1/2)*dq2*dqr1*cos(2*q5)*sin(q2)*sin(q3)*sin(q4))/4000000 + (1369*3^(1/2)*dq2*dqr1*sin(2*q5)*cos(q4)*sin(q2)*sin(q3))/8000000 - (1369*3^(1/2)*dq3*dqr1*cos(2*q5)*sin(q2)*sin(q3)*sin(q4))/4000000 - (1369*3^(1/2)*dq3*dqr1*sin(2*q5)*cos(q4)*sin(q2)*sin(q3))/8000000 - (1369*3^(1/2)*dq4*dqr1*sin(2*q5)*cos(q2)*sin(q3)*sin(q4))/8000000 + (1369*3^(1/2)*dq4*dqr1*sin(2*q5)*cos(q3)*sin(q2)*sin(q4))/8000000 + dq1*dqr1*cos(2*q2)*sin(2*q3)*sin(q4)*sin(q5)*((1369*3^(1/2))/4000000 - 45547/40000000) - dq1*dqr1*cos(2*q3)*sin(2*q2)*sin(q4)*sin(q5)*((1369*3^(1/2))/4000000 - 45547/40000000) + dq4*dqr1*cos(q2)*sin(q3)*sin(q4)*sin(q5)*((1369*3^(1/2))/2000000 + 71151/40000000) - dq4*dqr1*cos(q3)*sin(q2)*sin(q4)*sin(q5)*((1369*3^(1/2))/2000000 + 71151/40000000) + dq1*dqr1*cos(2*q2)*cos(2*q3)*sin(2*q4)*cos(q5)*((23717*3^(1/2))/80000000 + 1369/4000000) + dq1*dqr1*cos(2*q2)*cos(2*q3)*cos(2*q4)*sin(q5)*((23717*3^(1/2))/160000000 + 1369/8000000) + dq1*dqr1*sin(2*q2)*sin(2*q3)*sin(2*q4)*cos(q5)*((23717*3^(1/2))/80000000 + 1369/4000000) + dq1*dqr1*cos(2*q4)*sin(2*q2)*sin(2*q3)*sin(q5)*((23717*3^(1/2))/160000000 + 1369/8000000);
Y5_5_2=(4107*dq2*dqr2*sin(2*q5))/16000000 - (4107*dq2*dqr3*sin(2*q5))/16000000 - (4107*dq3*dqr2*sin(2*q5))/16000000 + (4107*dq3*dqr3*sin(2*q5))/16000000 - (4107*dq4*dqr4*sin(2*q5))/8000000 - dq4*dqr4*sin(q5)*((23717*3^(1/2))/40000000 + 1369/2000000) + dq2*dqr2*sin(q5)*((300773*3^(1/2))/80000000 - 1369/4000000) - dq2*dqr3*sin(q5)*((300773*3^(1/2))/80000000 - 1369/4000000) - dq3*dqr2*sin(q5)*((300773*3^(1/2))/80000000 - 1369/4000000) + dq3*dqr3*sin(q5)*((300773*3^(1/2))/80000000 - 1369/4000000) - (1369*3^(1/2)*dq2*dqr4*sin(q4))/4000000 - (1369*3^(1/2)*dq4*dqr2*sin(q4))/4000000 + (1369*3^(1/2)*dq3*dqr4*sin(q4))/4000000 + (1369*3^(1/2)*dq4*dqr3*sin(q4))/4000000 - (1369*dq2*dqr2*cos(2*q4)*sin(2*q5))/3200000 - (1369*dq2*dqr2*cos(2*q5)*sin(2*q4))/4000000 + (1369*dq2*dqr3*cos(2*q4)*sin(2*q5))/3200000 + (1369*dq2*dqr3*cos(2*q5)*sin(2*q4))/4000000 + (1369*dq3*dqr2*cos(2*q4)*sin(2*q5))/3200000 + (1369*dq3*dqr2*cos(2*q5)*sin(2*q4))/4000000 - (1369*dq3*dqr3*cos(2*q4)*sin(2*q5))/3200000 - (1369*dq3*dqr3*cos(2*q5)*sin(2*q4))/4000000 + (1369*dq1*dqr2*cos(q2)*sin(q3))/4000000 - (1369*dq1*dqr2*cos(q3)*sin(q2))/4000000 - (1369*dq1*dqr3*cos(q2)*sin(q3))/4000000 + (1369*dq1*dqr3*cos(q3)*sin(q2))/4000000 - dq2*dqr4*cos(q4)*sin(q5)*((1369*3^(1/2))/2000000 + 71151/40000000) - dq4*dqr2*cos(q4)*sin(q5)*((1369*3^(1/2))/2000000 + 71151/40000000) + dq3*dqr4*cos(q4)*sin(q5)*((1369*3^(1/2))/2000000 + 71151/40000000) + dq4*dqr3*cos(q4)*sin(q5)*((1369*3^(1/2))/2000000 + 71151/40000000) - (4107*dq1*dqr4*sin(2*q5)*cos(q2)*cos(q3))/8000000 - (4107*dq1*dqr4*sin(2*q5)*sin(q2)*sin(q3))/8000000 + (259*ddqr1*cos(q4)*cos(q5)*sin(q2)*sin(q3))/1000000 - (1073*3^(1/2)*dq2*dqr2*cos(q3)*sin(q5))/200000 - (259*ddqr1*sin(q2)*sin(q3)*sin(q4)*sin(q5))/2000000 + dq2*dqr2*sin(2*q4)*cos(q5)*((23717*3^(1/2))/40000000 + 1369/2000000) - dq2*dqr3*sin(2*q4)*cos(q5)*((23717*3^(1/2))/40000000 + 1369/2000000) - dq3*dqr2*sin(2*q4)*cos(q5)*((23717*3^(1/2))/40000000 + 1369/2000000) + dq3*dqr3*sin(2*q4)*cos(q5)*((23717*3^(1/2))/40000000 + 1369/2000000) + dq2*dqr2*cos(2*q4)*sin(q5)*((23717*3^(1/2))/80000000 + 1369/4000000) - dq2*dqr3*cos(2*q4)*sin(q5)*((23717*3^(1/2))/80000000 + 1369/4000000) - dq3*dqr2*cos(2*q4)*sin(q5)*((23717*3^(1/2))/80000000 + 1369/4000000) + dq3*dqr3*cos(2*q4)*sin(q5)*((23717*3^(1/2))/80000000 + 1369/4000000) + (1369*3^(1/2)*dq2*dqr4*cos(2*q5)*sin(q4))/4000000 + (1369*3^(1/2)*dq2*dqr4*sin(2*q5)*cos(q4))/8000000 + (1369*3^(1/2)*dq4*dqr2*cos(2*q5)*sin(q4))/4000000 + (1369*3^(1/2)*dq4*dqr2*sin(2*q5)*cos(q4))/8000000 - (1369*3^(1/2)*dq3*dqr4*cos(2*q5)*sin(q4))/4000000 - (1369*3^(1/2)*dq3*dqr4*sin(2*q5)*cos(q4))/8000000 - (1369*3^(1/2)*dq4*dqr3*cos(2*q5)*sin(q4))/4000000 - (1369*3^(1/2)*dq4*dqr3*sin(2*q5)*cos(q4))/8000000 - (1073*dq1*dqr2*cos(q2)*cos(q4)*sin(q5))/200000 - (1073*dq1*dqr2*cos(q2)*cos(q5)*sin(q4))/100000 + (1073*dq2*dqr2*cos(q4)*cos(q5)*sin(q3))/100000 - (1073*dq2*dqr2*sin(q3)*sin(q4)*sin(q5))/200000 + (1369*3^(1/2)*dq1*dqr2*cos(q2)*cos(q3)*sin(q4))/4000000 - (1369*3^(1/2)*dq1*dqr3*cos(q2)*cos(q3)*sin(q4))/4000000 - (1369*3^(1/2)*dq1*dqr4*cos(q2)*cos(q4)*sin(q3))/4000000 + (1369*3^(1/2)*dq1*dqr4*cos(q3)*cos(q4)*sin(q2))/4000000 - (1369*3^(1/2)*dq1*dqr3*sin(q2)*sin(q3)*sin(q4))/4000000 - (1369*dq1*dqr2*cos(2*q4)*cos(2*q5)*cos(q2)*sin(q3))/4000000 + (1369*dq1*dqr2*cos(2*q4)*cos(2*q5)*cos(q3)*sin(q2))/4000000 + (1369*dq1*dqr3*cos(2*q4)*cos(2*q5)*cos(q2)*sin(q3))/4000000 - (1369*dq1*dqr3*cos(2*q4)*cos(2*q5)*cos(q3)*sin(q2))/4000000 + (1369*dq1*dqr2*sin(2*q4)*sin(2*q5)*cos(q2)*sin(q3))/3200000 - (1369*dq1*dqr2*sin(2*q4)*sin(2*q5)*cos(q3)*sin(q2))/3200000 - (1369*dq1*dqr3*sin(2*q4)*sin(2*q5)*cos(q2)*sin(q3))/3200000 + (1369*dq1*dqr3*sin(2*q4)*sin(2*q5)*cos(q3)*sin(q2))/3200000 + (32449*dq1*dqr2*cos(q2)*cos(q3)*cos(q4)*sin(q5))/8000000 + (32449*dq1*dqr2*cos(q2)*cos(q3)*cos(q5)*sin(q4))/4000000 - (32449*dq1*dqr3*cos(q2)*cos(q3)*cos(q4)*sin(q5))/8000000 - (32449*dq1*dqr3*cos(q2)*cos(q3)*cos(q5)*sin(q4))/4000000 - (32449*dq1*dqr3*cos(q4)*sin(q2)*sin(q3)*sin(q5))/8000000 - (32449*dq1*dqr3*cos(q5)*sin(q2)*sin(q3)*sin(q4))/4000000 - dq1*dqr2*cos(q2)*cos(q5)*sin(q3)*((23717*3^(1/2))/40000000 + 1369/2000000) + dq1*dqr2*cos(q3)*cos(q5)*sin(q2)*((23717*3^(1/2))/40000000 + 1369/2000000) + dq1*dqr3*cos(q2)*cos(q5)*sin(q3)*((23717*3^(1/2))/40000000 + 1369/2000000) - dq1*dqr3*cos(q3)*cos(q5)*sin(q2)*((23717*3^(1/2))/40000000 + 1369/2000000) - dq1*dqr4*cos(q2)*cos(q3)*sin(q5)*((23717*3^(1/2))/40000000 + 1369/2000000) - dq1*dqr4*sin(q2)*sin(q3)*sin(q5)*((23717*3^(1/2))/40000000 + 1369/2000000) + dq1*dqr2*cos(2*q4)*cos(q2)*cos(q5)*sin(q3)*((23717*3^(1/2))/40000000 + 1369/2000000) - dq1*dqr2*cos(2*q4)*cos(q3)*cos(q5)*sin(q2)*((23717*3^(1/2))/40000000 + 1369/2000000) - dq1*dqr3*cos(2*q4)*cos(q2)*cos(q5)*sin(q3)*((23717*3^(1/2))/40000000 + 1369/2000000) + dq1*dqr3*cos(2*q4)*cos(q3)*cos(q5)*sin(q2)*((23717*3^(1/2))/40000000 + 1369/2000000) - dq1*dqr2*sin(2*q4)*cos(q2)*sin(q3)*sin(q5)*((23717*3^(1/2))/80000000 + 1369/4000000) + dq1*dqr2*sin(2*q4)*cos(q3)*sin(q2)*sin(q5)*((23717*3^(1/2))/80000000 + 1369/4000000) + dq1*dqr3*sin(2*q4)*cos(q2)*sin(q3)*sin(q5)*((23717*3^(1/2))/80000000 + 1369/4000000) - dq1*dqr3*sin(2*q4)*cos(q3)*sin(q2)*sin(q5)*((23717*3^(1/2))/80000000 + 1369/4000000) + (1369*3^(1/2)*dq1*dqr2*cos(2*q5)*cos(q2)*cos(q3)*sin(q4))/4000000 + (1369*3^(1/2)*dq1*dqr2*sin(2*q5)*cos(q2)*cos(q3)*cos(q4))/8000000 - (1369*3^(1/2)*dq1*dqr3*cos(2*q5)*cos(q2)*cos(q3)*sin(q4))/4000000 - (1369*3^(1/2)*dq1*dqr3*sin(2*q5)*cos(q2)*cos(q3)*cos(q4))/8000000 + (1369*3^(1/2)*dq1*dqr4*cos(2*q5)*cos(q2)*cos(q4)*sin(q3))/4000000 - (1369*3^(1/2)*dq1*dqr4*cos(2*q5)*cos(q3)*cos(q4)*sin(q2))/4000000 - (1369*3^(1/2)*dq1*dqr3*cos(2*q5)*sin(q2)*sin(q3)*sin(q4))/4000000 - (1369*3^(1/2)*dq1*dqr3*sin(2*q5)*cos(q4)*sin(q2)*sin(q3))/8000000 - (1369*3^(1/2)*dq1*dqr4*sin(2*q5)*cos(q2)*sin(q3)*sin(q4))/8000000 + (1369*3^(1/2)*dq1*dqr4*sin(2*q5)*cos(q3)*sin(q2)*sin(q4))/8000000 + dq1*dqr4*cos(q2)*sin(q3)*sin(q4)*sin(q5)*((1369*3^(1/2))/2000000 + 71151/40000000) - dq1*dqr4*cos(q3)*sin(q2)*sin(q4)*sin(q5)*((1369*3^(1/2))/2000000 + 71151/40000000);
Y5_5_3=(1369*ddqr4)/2000000 + (1369*ddqr5)/1000000 + (1369*ddqr1*cos(q2)*cos(q3))/2000000 + (32449*ddqr2*cos(q4)*cos(q5))/4000000 - (32449*ddqr3*cos(q4)*cos(q5))/4000000 + (1369*ddqr1*sin(q2)*sin(q3))/2000000 - ddqr4*cos(q5)*((23717*3^(1/2))/20000000 + 1369/1000000) + (1369*3^(1/2)*ddqr2*cos(q4))/2000000 - (1369*3^(1/2)*ddqr3*cos(q4))/2000000 - (1073*ddqr2*cos(q3)*cos(q4)*cos(q5))/100000 - (1073*ddqr1*cos(q4)*sin(q2)*sin(q5))/200000 - (1073*ddqr1*cos(q5)*sin(q2)*sin(q4))/100000 + (1073*ddqr2*cos(q3)*sin(q4)*sin(q5))/200000 - ddqr2*sin(q4)*sin(q5)*((1369*3^(1/2))/2000000 + 58349/10000000) + ddqr3*sin(q4)*sin(q5)*((1369*3^(1/2))/2000000 + 58349/10000000) - (1073*3^(1/2)*ddqr2*sin(q3)*sin(q5))/200000 + (259*ddqr1*cos(q2)*cos(q3)*cos(q4)*cos(q5))/1000000 - (259*ddqr1*cos(q2)*cos(q3)*sin(q4)*sin(q5))/2000000 - (32449*ddqr1*cos(q2)*cos(q5)*sin(q3)*sin(q4))/4000000 + (32449*ddqr1*cos(q3)*cos(q5)*sin(q2)*sin(q4))/4000000 - ddqr1*cos(q2)*cos(q3)*cos(q5)*((23717*3^(1/2))/20000000 + 1369/1000000) - ddqr1*cos(q5)*sin(q2)*sin(q3)*((23717*3^(1/2))/20000000 + 1369/1000000) - (1369*3^(1/2)*ddqr1*cos(q2)*sin(q3)*sin(q4))/2000000 + (1369*3^(1/2)*ddqr1*cos(q3)*sin(q2)*sin(q4))/2000000 + (259*3^(1/2)*ddqr1*cos(q2)*sin(q3)*sin(q5))/2000000 - (259*3^(1/2)*ddqr1*cos(q3)*sin(q2)*sin(q5))/2000000 - ddqr1*cos(q2)*cos(q4)*sin(q3)*sin(q5)*((1369*3^(1/2))/2000000 + 58349/10000000) + ddqr1*cos(q3)*cos(q4)*sin(q2)*sin(q5)*((1369*3^(1/2))/2000000 + 58349/10000000);
Y5_10_1=dq1*dqr1*sin(q5)*((259*3^(1/2))/32000 - 20541/320000) + (111*3^(1/2)*dq1*dqr1*sin(2*q5))/32000 + (87*dq1*dqr1*cos(q3)*sin(q5))/800 - (87*dq1*dqr1*cos(2*q2)*cos(q3)*sin(q5))/800 - (87*dq1*dqr1*sin(2*q2)*sin(q3)*sin(q5))/800 - (37*3^(1/2)*dq2*dqr1*cos(q2)*sin(q3))/4000 + (37*3^(1/2)*dq2*dqr1*cos(q3)*sin(q2))/4000 + (37*3^(1/2)*dq3*dqr1*cos(q2)*sin(q3))/4000 - (37*3^(1/2)*dq3*dqr1*cos(q3)*sin(q2))/4000 - (7*3^(1/2)*dq1*dqr1*cos(q4)*sin(q5))/4000 - (7*3^(1/2)*dq1*dqr1*cos(q5)*sin(q4))/2000 + dq1*dqr1*sin(2*q4)*cos(q5)*((111*3^(1/2))/16000 + 1923/160000) + dq1*dqr1*cos(2*q4)*sin(q5)*((111*3^(1/2))/32000 + 1923/320000) - (111*dq2*dqr1*cos(q2)*cos(q3)*sin(q4))/4000 + (111*dq3*dqr1*cos(q2)*cos(q3)*sin(q4))/4000 + (111*dq4*dqr1*cos(q2)*cos(q4)*sin(q3))/4000 - (111*dq4*dqr1*cos(q3)*cos(q4)*sin(q2))/4000 - (111*dq1*dqr2*sin(q2)*sin(q3)*sin(q4))/4000 - (111*dq2*dqr1*sin(q2)*sin(q3)*sin(q4))/4000 + (111*dq3*dqr1*sin(q2)*sin(q3)*sin(q4))/4000 - (37*3^(1/2)*dq1*dqr1*cos(2*q4)*sin(2*q5))/6400 - (37*3^(1/2)*dq1*dqr1*cos(2*q5)*sin(2*q4))/8000 - (111*dq1*dqr2*cos(2*q5)*sin(q2)*sin(q3)*sin(q4))/4000 - (111*dq1*dqr2*sin(2*q5)*cos(q4)*sin(q2)*sin(q3))/8000 - (111*dq2*dqr1*cos(2*q5)*sin(q2)*sin(q3)*sin(q4))/4000 - (111*dq2*dqr1*sin(2*q5)*cos(q4)*sin(q2)*sin(q3))/8000 + (111*dq3*dqr1*cos(2*q5)*sin(q2)*sin(q3)*sin(q4))/4000 + (111*dq3*dqr1*sin(2*q5)*cos(q4)*sin(q2)*sin(q3))/8000 + (111*dq4*dqr1*sin(2*q5)*cos(q2)*sin(q3)*sin(q4))/8000 - (111*dq4*dqr1*sin(2*q5)*cos(q3)*sin(q2)*sin(q4))/8000 - (29*3^(1/2)*dq1*dqr1*cos(q4)*cos(q5)*sin(q3))/400 + (29*3^(1/2)*dq2*dqr1*cos(q2)*cos(q4)*sin(q5))/400 + (29*3^(1/2)*dq2*dqr1*cos(q2)*cos(q5)*sin(q4))/200 + (333*3^(1/2)*dq1*dqr1*cos(2*q2)*cos(2*q3)*sin(2*q5))/32000 + (29*3^(1/2)*dq1*dqr1*sin(q3)*sin(q4)*sin(q5))/800 + (333*3^(1/2)*dq1*dqr1*sin(2*q2)*sin(2*q3)*sin(2*q5))/32000 + (111*3^(1/2)*dq4*dqr1*sin(2*q5)*cos(q2)*cos(q3))/8000 + dq1*dqr1*cos(2*q2)*cos(2*q3)*sin(q5)*((37*3^(1/2))/6400 + 28233/320000) + (111*3^(1/2)*dq4*dqr1*sin(2*q5)*sin(q2)*sin(q3))/8000 - (111*dq1*dqr1*cos(2*q2)*cos(2*q5)*sin(2*q3)*cos(q4))/4000 + (111*dq1*dqr1*cos(2*q3)*cos(2*q5)*sin(2*q2)*cos(q4))/4000 + dq1*dqr1*sin(2*q2)*sin(2*q3)*sin(q5)*((37*3^(1/2))/6400 + 28233/320000) + (111*dq1*dqr1*cos(2*q2)*sin(2*q3)*sin(2*q5)*sin(q4))/8000 - (111*dq1*dqr1*cos(2*q3)*sin(2*q2)*sin(2*q5)*sin(q4))/8000 + dq2*dqr1*cos(q2)*cos(q5)*sin(q3)*((111*3^(1/2))/8000 + 1923/80000) - dq2*dqr1*cos(q3)*cos(q5)*sin(q2)*((111*3^(1/2))/8000 + 1923/80000) - dq3*dqr1*cos(q2)*cos(q5)*sin(q3)*((111*3^(1/2))/8000 + 1923/80000) + dq3*dqr1*cos(q3)*cos(q5)*sin(q2)*((111*3^(1/2))/8000 + 1923/80000) + dq4*dqr1*cos(q2)*cos(q3)*sin(q5)*((111*3^(1/2))/8000 + 1923/80000) - (111*dq2*dqr1*cos(2*q5)*cos(q2)*cos(q3)*sin(q4))/4000 - (111*dq2*dqr1*sin(2*q5)*cos(q2)*cos(q3)*cos(q4))/8000 + (111*dq3*dqr1*cos(2*q5)*cos(q2)*cos(q3)*sin(q4))/4000 + (111*dq3*dqr1*sin(2*q5)*cos(q2)*cos(q3)*cos(q4))/8000 - (111*dq4*dqr1*cos(2*q5)*cos(q2)*cos(q4)*sin(q3))/4000 + (111*dq4*dqr1*cos(2*q5)*cos(q3)*cos(q4)*sin(q2))/4000 + dq4*dqr1*sin(q2)*sin(q3)*sin(q5)*((111*3^(1/2))/8000 + 1923/80000) - dq2*dqr1*cos(2*q4)*cos(q2)*cos(q5)*sin(q3)*((111*3^(1/2))/8000 + 1923/80000) + dq2*dqr1*cos(2*q4)*cos(q3)*cos(q5)*sin(q2)*((111*3^(1/2))/8000 + 1923/80000) + dq3*dqr1*cos(2*q4)*cos(q2)*cos(q5)*sin(q3)*((111*3^(1/2))/8000 + 1923/80000) - dq3*dqr1*cos(2*q4)*cos(q3)*cos(q5)*sin(q2)*((111*3^(1/2))/8000 + 1923/80000) + dq2*dqr1*sin(2*q4)*cos(q2)*sin(q3)*sin(q5)*((111*3^(1/2))/16000 + 1923/160000) - dq2*dqr1*sin(2*q4)*cos(q3)*sin(q2)*sin(q5)*((111*3^(1/2))/16000 + 1923/160000) - dq3*dqr1*sin(2*q4)*cos(q2)*sin(q3)*sin(q5)*((111*3^(1/2))/16000 + 1923/160000) + dq3*dqr1*sin(2*q4)*cos(q3)*sin(q2)*sin(q5)*((111*3^(1/2))/16000 + 1923/160000) + (29*3^(1/2)*dq1*dqr1*cos(2*q2)*cos(q4)*cos(q5)*sin(q3))/400 - (29*3^(1/2)*dq1*dqr1*sin(2*q2)*cos(q3)*cos(q4)*cos(q5))/400 + (37*3^(1/2)*dq1*dqr1*cos(2*q2)*cos(2*q3)*cos(2*q4)*sin(2*q5))/6400 + (37*3^(1/2)*dq1*dqr1*cos(2*q2)*cos(2*q3)*cos(2*q5)*sin(2*q4))/8000 - dq1*dqr1*cos(2*q2)*sin(2*q3)*cos(q4)*cos(q5)*((877*3^(1/2))/16000 + 37/8000) + dq1*dqr1*cos(2*q3)*sin(2*q2)*cos(q4)*cos(q5)*((877*3^(1/2))/16000 + 37/8000) - (29*3^(1/2)*dq1*dqr1*cos(2*q2)*sin(q3)*sin(q4)*sin(q5))/800 + (29*3^(1/2)*dq1*dqr1*sin(2*q2)*cos(q3)*sin(q4)*sin(q5))/800 + (37*3^(1/2)*dq1*dqr1*cos(2*q4)*sin(2*q2)*sin(2*q3)*sin(2*q5))/6400 + (37*3^(1/2)*dq1*dqr1*cos(2*q5)*sin(2*q2)*sin(2*q3)*sin(2*q4))/8000 + dq1*dqr1*cos(2*q2)*sin(2*q3)*sin(q4)*sin(q5)*((1231*3^(1/2))/80000 - 37/2000) - dq1*dqr1*cos(2*q3)*sin(2*q2)*sin(q4)*sin(q5)*((1231*3^(1/2))/80000 - 37/2000) + (37*3^(1/2)*dq2*dqr1*cos(2*q4)*cos(2*q5)*cos(q2)*sin(q3))/4000 - (37*3^(1/2)*dq2*dqr1*cos(2*q4)*cos(2*q5)*cos(q3)*sin(q2))/4000 - (37*3^(1/2)*dq3*dqr1*cos(2*q4)*cos(2*q5)*cos(q2)*sin(q3))/4000 + (37*3^(1/2)*dq3*dqr1*cos(2*q4)*cos(2*q5)*cos(q3)*sin(q2))/4000 - dq2*dqr1*cos(q2)*cos(q3)*cos(q5)*sin(q4)*((877*3^(1/2))/8000 + 37/4000) + dq3*dqr1*cos(q2)*cos(q3)*cos(q5)*sin(q4)*((877*3^(1/2))/8000 + 37/4000) - dq2*dqr1*cos(q2)*cos(q3)*cos(q4)*sin(q5)*((877*3^(1/2))/16000 + 37/8000) + dq3*dqr1*cos(q2)*cos(q3)*cos(q4)*sin(q5)*((877*3^(1/2))/16000 + 37/8000) - dq1*dqr1*cos(2*q2)*cos(2*q3)*sin(2*q4)*cos(q5)*((111*3^(1/2))/16000 + 1923/160000) - dq1*dqr1*cos(2*q2)*cos(2*q3)*cos(2*q4)*sin(q5)*((111*3^(1/2))/32000 + 1923/320000) - (37*3^(1/2)*dq2*dqr1*sin(2*q4)*sin(2*q5)*cos(q2)*sin(q3))/3200 + (37*3^(1/2)*dq2*dqr1*sin(2*q4)*sin(2*q5)*cos(q3)*sin(q2))/3200 + (37*3^(1/2)*dq3*dqr1*sin(2*q4)*sin(2*q5)*cos(q2)*sin(q3))/3200 - (37*3^(1/2)*dq3*dqr1*sin(2*q4)*sin(2*q5)*cos(q3)*sin(q2))/3200 - dq1*dqr2*cos(q5)*sin(q2)*sin(q3)*sin(q4)*((877*3^(1/2))/8000 + 37/4000) - dq2*dqr1*cos(q5)*sin(q2)*sin(q3)*sin(q4)*((877*3^(1/2))/8000 + 37/4000) + dq3*dqr1*cos(q5)*sin(q2)*sin(q3)*sin(q4)*((877*3^(1/2))/8000 + 37/4000) - dq1*dqr2*cos(q4)*sin(q2)*sin(q3)*sin(q5)*((877*3^(1/2))/16000 + 37/8000) - dq2*dqr1*cos(q4)*sin(q2)*sin(q3)*sin(q5)*((877*3^(1/2))/16000 + 37/8000) + dq3*dqr1*cos(q4)*sin(q2)*sin(q3)*sin(q5)*((877*3^(1/2))/16000 + 37/8000) - dq4*dqr1*cos(q2)*sin(q3)*sin(q4)*sin(q5)*((1923*3^(1/2))/80000 + 333/8000) + dq4*dqr1*cos(q3)*sin(q2)*sin(q4)*sin(q5)*((1923*3^(1/2))/80000 + 333/8000) - dq1*dqr1*sin(2*q2)*sin(2*q3)*sin(2*q4)*cos(q5)*((111*3^(1/2))/16000 + 1923/160000) - dq1*dqr1*cos(2*q4)*sin(2*q2)*sin(2*q3)*sin(q5)*((111*3^(1/2))/32000 + 1923/320000);
Y5_10_2=(111*dq2*dqr4*sin(q4))/4000 + (111*dq4*dqr2*sin(q4))/4000 - (111*dq3*dqr4*sin(q4))/4000 - (111*dq4*dqr3*sin(q4))/4000 + dq4*dqr4*sin(q5)*((111*3^(1/2))/8000 + 1923/80000) + dq2*dqr2*sin(q5)*((37*3^(1/2))/16000 - 24387/160000) - dq2*dqr3*sin(q5)*((37*3^(1/2))/16000 - 24387/160000) - dq3*dqr2*sin(q5)*((37*3^(1/2))/16000 - 24387/160000) + dq3*dqr3*sin(q5)*((37*3^(1/2))/16000 - 24387/160000) - (111*dq2*dqr4*cos(2*q5)*sin(q4))/4000 - (111*dq2*dqr4*sin(2*q5)*cos(q4))/8000 - (111*dq4*dqr2*cos(2*q5)*sin(q4))/4000 - (111*dq4*dqr2*sin(2*q5)*cos(q4))/8000 + (111*dq3*dqr4*cos(2*q5)*sin(q4))/4000 + (111*dq3*dqr4*sin(2*q5)*cos(q4))/8000 + (111*dq4*dqr3*cos(2*q5)*sin(q4))/4000 + (111*dq4*dqr3*sin(2*q5)*cos(q4))/8000 - (111*3^(1/2)*dq2*dqr2*sin(2*q5))/16000 + (111*3^(1/2)*dq2*dqr3*sin(2*q5))/16000 + (111*3^(1/2)*dq3*dqr2*sin(2*q5))/16000 - (111*3^(1/2)*dq3*dqr3*sin(2*q5))/16000 + (111*3^(1/2)*dq4*dqr4*sin(2*q5))/8000 + (87*dq2*dqr2*cos(q3)*sin(q5))/400 - (37*3^(1/2)*dq1*dqr2*cos(q2)*sin(q3))/4000 + (37*3^(1/2)*dq1*dqr2*cos(q3)*sin(q2))/4000 + (37*3^(1/2)*dq1*dqr3*cos(q2)*sin(q3))/4000 - (37*3^(1/2)*dq1*dqr3*cos(q3)*sin(q2))/4000 - dq2*dqr2*sin(2*q4)*cos(q5)*((111*3^(1/2))/8000 + 1923/80000) + dq2*dqr3*sin(2*q4)*cos(q5)*((111*3^(1/2))/8000 + 1923/80000) + dq3*dqr2*sin(2*q4)*cos(q5)*((111*3^(1/2))/8000 + 1923/80000) - dq3*dqr3*sin(2*q4)*cos(q5)*((111*3^(1/2))/8000 + 1923/80000) - dq2*dqr2*cos(2*q4)*sin(q5)*((111*3^(1/2))/16000 + 1923/160000) + dq2*dqr3*cos(2*q4)*sin(q5)*((111*3^(1/2))/16000 + 1923/160000) + dq3*dqr2*cos(2*q4)*sin(q5)*((111*3^(1/2))/16000 + 1923/160000) - dq3*dqr3*cos(2*q4)*sin(q5)*((111*3^(1/2))/16000 + 1923/160000) - (111*dq1*dqr2*cos(q2)*cos(q3)*sin(q4))/4000 + (111*dq1*dqr3*cos(q2)*cos(q3)*sin(q4))/4000 + (111*dq1*dqr4*cos(q2)*cos(q4)*sin(q3))/4000 - (111*dq1*dqr4*cos(q3)*cos(q4)*sin(q2))/4000 + (111*dq1*dqr3*sin(q2)*sin(q3)*sin(q4))/4000 + (37*3^(1/2)*dq2*dqr2*cos(2*q4)*sin(2*q5))/3200 + (37*3^(1/2)*dq2*dqr2*cos(2*q5)*sin(2*q4))/4000 - (37*3^(1/2)*dq2*dqr3*cos(2*q4)*sin(2*q5))/3200 - (37*3^(1/2)*dq2*dqr3*cos(2*q5)*sin(2*q4))/4000 - (37*3^(1/2)*dq3*dqr2*cos(2*q4)*sin(2*q5))/3200 - (37*3^(1/2)*dq3*dqr2*cos(2*q5)*sin(2*q4))/4000 + (37*3^(1/2)*dq3*dqr3*cos(2*q4)*sin(2*q5))/3200 + (37*3^(1/2)*dq3*dqr3*cos(2*q5)*sin(2*q4))/4000 + dq2*dqr4*cos(q4)*sin(q5)*((1923*3^(1/2))/80000 + 333/8000) + dq4*dqr2*cos(q4)*sin(q5)*((1923*3^(1/2))/80000 + 333/8000) - dq3*dqr4*cos(q4)*sin(q5)*((1923*3^(1/2))/80000 + 333/8000) - dq4*dqr3*cos(q4)*sin(q5)*((1923*3^(1/2))/80000 + 333/8000) + (111*dq1*dqr3*cos(2*q5)*sin(q2)*sin(q3)*sin(q4))/4000 + (111*dq1*dqr3*sin(2*q5)*cos(q4)*sin(q2)*sin(q3))/8000 + (111*dq1*dqr4*sin(2*q5)*cos(q2)*sin(q3)*sin(q4))/8000 - (111*dq1*dqr4*sin(2*q5)*cos(q3)*sin(q2)*sin(q4))/8000 + (29*3^(1/2)*dq1*dqr2*cos(q2)*cos(q4)*sin(q5))/400 + (29*3^(1/2)*dq1*dqr2*cos(q2)*cos(q5)*sin(q4))/200 - (29*3^(1/2)*dq2*dqr2*cos(q4)*cos(q5)*sin(q3))/200 + (29*3^(1/2)*dq2*dqr2*sin(q3)*sin(q4)*sin(q5))/400 + (111*3^(1/2)*dq1*dqr4*sin(2*q5)*cos(q2)*cos(q3))/8000 + (111*3^(1/2)*dq1*dqr4*sin(2*q5)*sin(q2)*sin(q3))/8000 - (7*3^(1/2)*ddqr1*cos(q4)*cos(q5)*sin(q2)*sin(q3))/2000 + (7*3^(1/2)*ddqr1*sin(q2)*sin(q3)*sin(q4)*sin(q5))/4000 + dq1*dqr2*cos(q2)*cos(q5)*sin(q3)*((111*3^(1/2))/8000 + 1923/80000) - dq1*dqr2*cos(q3)*cos(q5)*sin(q2)*((111*3^(1/2))/8000 + 1923/80000) - dq1*dqr3*cos(q2)*cos(q5)*sin(q3)*((111*3^(1/2))/8000 + 1923/80000) + dq1*dqr3*cos(q3)*cos(q5)*sin(q2)*((111*3^(1/2))/8000 + 1923/80000) + dq1*dqr4*cos(q2)*cos(q3)*sin(q5)*((111*3^(1/2))/8000 + 1923/80000) - (111*dq1*dqr2*cos(2*q5)*cos(q2)*cos(q3)*sin(q4))/4000 - (111*dq1*dqr2*sin(2*q5)*cos(q2)*cos(q3)*cos(q4))/8000 + (111*dq1*dqr3*cos(2*q5)*cos(q2)*cos(q3)*sin(q4))/4000 + (111*dq1*dqr3*sin(2*q5)*cos(q2)*cos(q3)*cos(q4))/8000 - (111*dq1*dqr4*cos(2*q5)*cos(q2)*cos(q4)*sin(q3))/4000 + (111*dq1*dqr4*cos(2*q5)*cos(q3)*cos(q4)*sin(q2))/4000 + dq1*dqr4*sin(q2)*sin(q3)*sin(q5)*((111*3^(1/2))/8000 + 1923/80000) - dq1*dqr2*cos(2*q4)*cos(q2)*cos(q5)*sin(q3)*((111*3^(1/2))/8000 + 1923/80000) + dq1*dqr2*cos(2*q4)*cos(q3)*cos(q5)*sin(q2)*((111*3^(1/2))/8000 + 1923/80000) + dq1*dqr3*cos(2*q4)*cos(q2)*cos(q5)*sin(q3)*((111*3^(1/2))/8000 + 1923/80000) - dq1*dqr3*cos(2*q4)*cos(q3)*cos(q5)*sin(q2)*((111*3^(1/2))/8000 + 1923/80000) + dq1*dqr2*sin(2*q4)*cos(q2)*sin(q3)*sin(q5)*((111*3^(1/2))/16000 + 1923/160000) - dq1*dqr2*sin(2*q4)*cos(q3)*sin(q2)*sin(q5)*((111*3^(1/2))/16000 + 1923/160000) - dq1*dqr3*sin(2*q4)*cos(q2)*sin(q3)*sin(q5)*((111*3^(1/2))/16000 + 1923/160000) + dq1*dqr3*sin(2*q4)*cos(q3)*sin(q2)*sin(q5)*((111*3^(1/2))/16000 + 1923/160000) + (37*3^(1/2)*dq1*dqr2*cos(2*q4)*cos(2*q5)*cos(q2)*sin(q3))/4000 - (37*3^(1/2)*dq1*dqr2*cos(2*q4)*cos(2*q5)*cos(q3)*sin(q2))/4000 - (37*3^(1/2)*dq1*dqr3*cos(2*q4)*cos(2*q5)*cos(q2)*sin(q3))/4000 + (37*3^(1/2)*dq1*dqr3*cos(2*q4)*cos(2*q5)*cos(q3)*sin(q2))/4000 - dq1*dqr2*cos(q2)*cos(q3)*cos(q5)*sin(q4)*((877*3^(1/2))/8000 + 37/4000) + dq1*dqr3*cos(q2)*cos(q3)*cos(q5)*sin(q4)*((877*3^(1/2))/8000 + 37/4000) - dq1*dqr2*cos(q2)*cos(q3)*cos(q4)*sin(q5)*((877*3^(1/2))/16000 + 37/8000) + dq1*dqr3*cos(q2)*cos(q3)*cos(q4)*sin(q5)*((877*3^(1/2))/16000 + 37/8000) - (37*3^(1/2)*dq1*dqr2*sin(2*q4)*sin(2*q5)*cos(q2)*sin(q3))/3200 + (37*3^(1/2)*dq1*dqr2*sin(2*q4)*sin(2*q5)*cos(q3)*sin(q2))/3200 + (37*3^(1/2)*dq1*dqr3*sin(2*q4)*sin(2*q5)*cos(q2)*sin(q3))/3200 - (37*3^(1/2)*dq1*dqr3*sin(2*q4)*sin(2*q5)*cos(q3)*sin(q2))/3200 + dq1*dqr3*cos(q5)*sin(q2)*sin(q3)*sin(q4)*((877*3^(1/2))/8000 + 37/4000) + dq1*dqr3*cos(q4)*sin(q2)*sin(q3)*sin(q5)*((877*3^(1/2))/16000 + 37/8000) - dq1*dqr4*cos(q2)*sin(q3)*sin(q4)*sin(q5)*((1923*3^(1/2))/80000 + 333/8000) + dq1*dqr4*cos(q3)*sin(q2)*sin(q4)*sin(q5)*((1923*3^(1/2))/80000 + 333/8000);
Y5_10_3=(111*ddqr3*cos(q4))/2000 - (37*3^(1/2)*ddqr5)/1000 - (111*ddqr2*cos(q4))/2000 - (37*3^(1/2)*ddqr4)/2000 + (87*ddqr2*sin(q3)*sin(q5))/400 + ddqr4*cos(q5)*((111*3^(1/2))/4000 + 1923/40000) + (111*ddqr1*cos(q2)*sin(q3)*sin(q4))/2000 - (111*ddqr1*cos(q3)*sin(q2)*sin(q4))/2000 - (21*ddqr1*cos(q2)*sin(q3)*sin(q5))/4000 + (21*ddqr1*cos(q3)*sin(q2)*sin(q5))/4000 - ddqr2*cos(q4)*cos(q5)*((877*3^(1/2))/8000 + 37/4000) + ddqr3*cos(q4)*cos(q5)*((877*3^(1/2))/8000 + 37/4000) + ddqr2*sin(q4)*sin(q5)*((1577*3^(1/2))/20000 + 37/800) - ddqr3*sin(q4)*sin(q5)*((1577*3^(1/2))/20000 + 37/800) - (37*3^(1/2)*ddqr1*cos(q2)*cos(q3))/2000 - (37*3^(1/2)*ddqr1*sin(q2)*sin(q3))/2000 + ddqr1*cos(q2)*cos(q3)*cos(q5)*((111*3^(1/2))/4000 + 1923/40000) + ddqr1*cos(q5)*sin(q2)*sin(q3)*((111*3^(1/2))/4000 + 1923/40000) + (29*3^(1/2)*ddqr2*cos(q3)*cos(q4)*cos(q5))/200 + (29*3^(1/2)*ddqr1*cos(q4)*sin(q2)*sin(q5))/400 + (29*3^(1/2)*ddqr1*cos(q5)*sin(q2)*sin(q4))/200 - (29*3^(1/2)*ddqr2*cos(q3)*sin(q4)*sin(q5))/400 + ddqr1*cos(q2)*cos(q5)*sin(q3)*sin(q4)*((877*3^(1/2))/8000 + 37/4000) - ddqr1*cos(q3)*cos(q5)*sin(q2)*sin(q4)*((877*3^(1/2))/8000 + 37/4000) + ddqr1*cos(q2)*cos(q4)*sin(q3)*sin(q5)*((1577*3^(1/2))/20000 + 37/800) - ddqr1*cos(q3)*cos(q4)*sin(q2)*sin(q5)*((1577*3^(1/2))/20000 + 37/800) - (7*3^(1/2)*ddqr1*cos(q2)*cos(q3)*cos(q4)*cos(q5))/2000 + (7*3^(1/2)*ddqr1*cos(q2)*cos(q3)*sin(q4)*sin(q5))/4000;
Y5_14_1=(37*cos(q2)*cos(q4)*cos(q5)*sin(q3))/1000 - (37*3^(1/2)*sin(q2)*sin(q3)*sin(q5))/2000 - (37*3^(1/2)*cos(q2)*cos(q3)*sin(q5))/2000 - (37*cos(q3)*cos(q4)*cos(q5)*sin(q2))/1000 - (37*cos(q2)*sin(q3)*sin(q4)*sin(q5))/2000 + (37*cos(q3)*sin(q2)*sin(q4)*sin(q5))/2000;
Y5_19_1=(15*dq1*dqr1*cos(2*q4)*sin(2*q5))/128 - (9*dq1*dqr1*sin(2*q5))/128 - (3*dq1*dqr1*cos(2*q4)*sin(q5))/64 - (3*dq1*dqr1*sin(2*q4)*cos(q5))/32 - (3*dq1*dqr1*sin(q5))/64 + (3*dq1*dqr1*cos(2*q5)*sin(2*q4))/32 + (3*dq1*dqr2*cos(q2)*sin(q3))/16 - (3*dq1*dqr2*cos(q3)*sin(q2))/16 + (3*dq2*dqr1*cos(q2)*sin(q3))/16 - (3*dq2*dqr1*cos(q3)*sin(q2))/16 - (3*dq3*dqr1*cos(q2)*sin(q3))/16 + (3*dq3*dqr1*cos(q3)*sin(q2))/16 - (9*dq4*dqr1*sin(2*q5)*cos(q2)*cos(q3))/32 - (9*dq4*dqr1*sin(2*q5)*sin(q2)*sin(q3))/32 - (9*dq1*dqr1*cos(2*q2)*cos(2*q3)*sin(q5))/64 - (9*dq1*dqr1*sin(2*q2)*sin(2*q3)*sin(q5))/64 - (3*dq1*dqr2*cos(q2)*cos(q5)*sin(q3))/16 + (3*dq1*dqr2*cos(q3)*cos(q5)*sin(q2))/16 - (3*dq2*dqr1*cos(q2)*cos(q5)*sin(q3))/16 + (3*dq2*dqr1*cos(q3)*cos(q5)*sin(q2))/16 + (3*dq3*dqr1*cos(q2)*cos(q5)*sin(q3))/16 - (3*dq3*dqr1*cos(q3)*cos(q5)*sin(q2))/16 - (3*dq4*dqr1*cos(q2)*cos(q3)*sin(q5))/16 - (27*dq1*dqr1*cos(2*q2)*cos(2*q3)*sin(2*q5))/128 - (3*dq4*dqr1*sin(q2)*sin(q3)*sin(q5))/16 - (27*dq1*dqr1*sin(2*q2)*sin(2*q3)*sin(2*q5))/128 - (15*dq1*dqr1*cos(2*q2)*cos(2*q3)*cos(2*q4)*sin(2*q5))/128 - (3*dq1*dqr1*cos(2*q2)*cos(2*q3)*cos(2*q5)*sin(2*q4))/32 - (3*dq1*dqr2*sin(2*q4)*cos(q2)*sin(q3)*sin(q5))/32 + (3*dq1*dqr2*sin(2*q4)*cos(q3)*sin(q2)*sin(q5))/32 - (3*dq2*dqr1*sin(2*q4)*cos(q2)*sin(q3)*sin(q5))/32 + (3*dq2*dqr1*sin(2*q4)*cos(q3)*sin(q2)*sin(q5))/32 + (3*dq3*dqr1*sin(2*q4)*cos(q2)*sin(q3)*sin(q5))/32 - (3*dq3*dqr1*sin(2*q4)*cos(q3)*sin(q2)*sin(q5))/32 + (3*3^(1/2)*dq2*dqr1*cos(q2)*cos(q3)*sin(q4))/16 - (3*3^(1/2)*dq3*dqr1*cos(q2)*cos(q3)*sin(q4))/16 - (3*3^(1/2)*dq4*dqr1*cos(q2)*cos(q4)*sin(q3))/16 + (3*3^(1/2)*dq4*dqr1*cos(q3)*cos(q4)*sin(q2))/16 - (15*dq1*dqr1*cos(2*q4)*sin(2*q2)*sin(2*q3)*sin(2*q5))/128 - (3*dq1*dqr1*cos(2*q5)*sin(2*q2)*sin(2*q3)*sin(2*q4))/32 + (3*3^(1/2)*dq1*dqr2*sin(q2)*sin(q3)*sin(q4))/16 + (3*3^(1/2)*dq2*dqr1*sin(q2)*sin(q3)*sin(q4))/16 - (3*3^(1/2)*dq3*dqr1*sin(q2)*sin(q3)*sin(q4))/16 - (3*dq1*dqr2*cos(2*q4)*cos(2*q5)*cos(q2)*sin(q3))/16 + (3*dq1*dqr2*cos(2*q4)*cos(2*q5)*cos(q3)*sin(q2))/16 - (3*dq2*dqr1*cos(2*q4)*cos(2*q5)*cos(q2)*sin(q3))/16 + (3*dq2*dqr1*cos(2*q4)*cos(2*q5)*cos(q3)*sin(q2))/16 + (3*dq3*dqr1*cos(2*q4)*cos(2*q5)*cos(q2)*sin(q3))/16 - (3*dq3*dqr1*cos(2*q4)*cos(2*q5)*cos(q3)*sin(q2))/16 + (15*dq1*dqr2*sin(2*q4)*sin(2*q5)*cos(q2)*sin(q3))/64 - (15*dq1*dqr2*sin(2*q4)*sin(2*q5)*cos(q3)*sin(q2))/64 + (15*dq2*dqr1*sin(2*q4)*sin(2*q5)*cos(q2)*sin(q3))/64 - (15*dq2*dqr1*sin(2*q4)*sin(2*q5)*cos(q3)*sin(q2))/64 - (15*dq3*dqr1*sin(2*q4)*sin(2*q5)*cos(q2)*sin(q3))/64 + (15*dq3*dqr1*sin(2*q4)*sin(2*q5)*cos(q3)*sin(q2))/64 + (3*dq1*dqr1*cos(2*q2)*cos(2*q3)*cos(2*q4)*sin(q5))/64 + (3*dq1*dqr1*cos(2*q2)*cos(2*q3)*sin(2*q4)*cos(q5))/32 + (3*dq1*dqr1*cos(2*q4)*sin(2*q2)*sin(2*q3)*sin(q5))/64 + (3*dq1*dqr1*sin(2*q2)*sin(2*q3)*sin(2*q4)*cos(q5))/32 + (3*dq1*dqr2*cos(2*q4)*cos(q2)*cos(q5)*sin(q3))/16 - (3*dq1*dqr2*cos(2*q4)*cos(q3)*cos(q5)*sin(q2))/16 + (3*dq2*dqr1*cos(2*q4)*cos(q2)*cos(q5)*sin(q3))/16 - (3*dq2*dqr1*cos(2*q4)*cos(q3)*cos(q5)*sin(q2))/16 - (3*dq3*dqr1*cos(2*q4)*cos(q2)*cos(q5)*sin(q3))/16 + (3*dq3*dqr1*cos(2*q4)*cos(q3)*cos(q5)*sin(q2))/16 + (3*3^(1/2)*dq1*dqr1*cos(2*q2)*cos(2*q5)*sin(2*q3)*cos(q4))/16 - (3*3^(1/2)*dq1*dqr1*cos(2*q3)*cos(2*q5)*sin(2*q2)*cos(q4))/16 + (3^(1/2)*dq1*dqr2*cos(q4)*sin(q2)*sin(q3)*sin(q5))/16 + (3^(1/2)*dq1*dqr2*cos(q5)*sin(q2)*sin(q3)*sin(q4))/8 + (3^(1/2)*dq2*dqr1*cos(q4)*sin(q2)*sin(q3)*sin(q5))/16 + (3^(1/2)*dq2*dqr1*cos(q5)*sin(q2)*sin(q3)*sin(q4))/8 - (3^(1/2)*dq3*dqr1*cos(q4)*sin(q2)*sin(q3)*sin(q5))/16 - (3^(1/2)*dq3*dqr1*cos(q5)*sin(q2)*sin(q3)*sin(q4))/8 + (3*3^(1/2)*dq4*dqr1*cos(q2)*sin(q3)*sin(q4)*sin(q5))/16 - (3*3^(1/2)*dq4*dqr1*cos(q3)*sin(q2)*sin(q4)*sin(q5))/16 - (3*3^(1/2)*dq1*dqr1*cos(2*q2)*sin(2*q3)*sin(2*q5)*sin(q4))/32 + (3*3^(1/2)*dq1*dqr1*cos(2*q3)*sin(2*q2)*sin(2*q5)*sin(q4))/32 + (3*3^(1/2)*dq2*dqr1*cos(2*q5)*cos(q2)*cos(q3)*sin(q4))/16 + (3*3^(1/2)*dq2*dqr1*sin(2*q5)*cos(q2)*cos(q3)*cos(q4))/32 - (3*3^(1/2)*dq3*dqr1*cos(2*q5)*cos(q2)*cos(q3)*sin(q4))/16 - (3*3^(1/2)*dq3*dqr1*sin(2*q5)*cos(q2)*cos(q3)*cos(q4))/32 + (3*3^(1/2)*dq4*dqr1*cos(2*q5)*cos(q2)*cos(q4)*sin(q3))/16 - (3*3^(1/2)*dq4*dqr1*cos(2*q5)*cos(q3)*cos(q4)*sin(q2))/16 + (3*3^(1/2)*dq1*dqr2*cos(2*q5)*sin(q2)*sin(q3)*sin(q4))/16 + (3*3^(1/2)*dq1*dqr2*sin(2*q5)*cos(q4)*sin(q2)*sin(q3))/32 + (3*3^(1/2)*dq2*dqr1*cos(2*q5)*sin(q2)*sin(q3)*sin(q4))/16 + (3*3^(1/2)*dq2*dqr1*sin(2*q5)*cos(q4)*sin(q2)*sin(q3))/32 - (3*3^(1/2)*dq3*dqr1*cos(2*q5)*sin(q2)*sin(q3)*sin(q4))/16 - (3*3^(1/2)*dq3*dqr1*sin(2*q5)*cos(q4)*sin(q2)*sin(q3))/32 - (3*3^(1/2)*dq4*dqr1*sin(2*q5)*cos(q2)*sin(q3)*sin(q4))/32 + (3*3^(1/2)*dq4*dqr1*sin(2*q5)*cos(q3)*sin(q2)*sin(q4))/32 + (3^(1/2)*dq1*dqr1*cos(2*q2)*sin(2*q3)*cos(q4)*cos(q5))/16 - (3^(1/2)*dq1*dqr1*cos(2*q3)*sin(2*q2)*cos(q4)*cos(q5))/16 + (3^(1/2)*dq1*dqr1*cos(2*q2)*sin(2*q3)*sin(q4)*sin(q5))/16 - (3^(1/2)*dq1*dqr1*cos(2*q3)*sin(2*q2)*sin(q4)*sin(q5))/16 + (3^(1/2)*dq1*dqr2*cos(q2)*cos(q3)*cos(q5)*sin(q4))/8 + (3^(1/2)*dq2*dqr1*cos(q2)*cos(q3)*cos(q4)*sin(q5))/16 + (3^(1/2)*dq2*dqr1*cos(q2)*cos(q3)*cos(q5)*sin(q4))/8 - (3^(1/2)*dq3*dqr1*cos(q2)*cos(q3)*cos(q4)*sin(q5))/16 - (3^(1/2)*dq3*dqr1*cos(q2)*cos(q3)*cos(q5)*sin(q4))/8;
Y5_19_2=(3*ddqr4)/8 + (3*ddqr5)/4 - (3*ddqr4*cos(q5))/8 + (3*dq2*dqr2*sin(q5))/32 - (3*dq2*dqr3*sin(q5))/32 - (3*dq3*dqr2*sin(q5))/32 + (3*dq3*dqr3*sin(q5))/32 - (3*dq4*dqr4*sin(q5))/16 + (9*dq2*dqr2*sin(2*q5))/64 - (9*dq2*dqr3*sin(2*q5))/64 - (9*dq3*dqr2*sin(2*q5))/64 + (9*dq3*dqr3*sin(2*q5))/64 - (9*dq4*dqr4*sin(2*q5))/32 + (3*ddqr1*cos(q2)*cos(q3))/8 + (3*ddqr1*sin(q2)*sin(q3))/8 + (3*3^(1/2)*ddqr2*cos(q4))/8 - (3*3^(1/2)*ddqr3*cos(q4))/8 + (3*dq2*dqr2*cos(2*q4)*sin(q5))/32 + (3*dq2*dqr2*sin(2*q4)*cos(q5))/16 - (3*dq2*dqr3*cos(2*q4)*sin(q5))/32 - (3*dq2*dqr3*sin(2*q4)*cos(q5))/16 - (3*dq3*dqr2*cos(2*q4)*sin(q5))/32 - (3*dq3*dqr2*sin(2*q4)*cos(q5))/16 + (3*dq3*dqr3*cos(2*q4)*sin(q5))/32 + (3*dq3*dqr3*sin(2*q4)*cos(q5))/16 - (3*ddqr1*cos(q2)*cos(q3)*cos(q5))/8 - (3*ddqr1*cos(q5)*sin(q2)*sin(q3))/8 - (3*3^(1/2)*dq2*dqr4*sin(q4))/16 - (3*3^(1/2)*dq4*dqr2*sin(q4))/16 + (3*3^(1/2)*dq3*dqr4*sin(q4))/16 + (3*3^(1/2)*dq4*dqr3*sin(q4))/16 - (15*dq2*dqr2*cos(2*q4)*sin(2*q5))/64 - (3*dq2*dqr2*cos(2*q5)*sin(2*q4))/16 + (15*dq2*dqr3*cos(2*q4)*sin(2*q5))/64 + (3*dq2*dqr3*cos(2*q5)*sin(2*q4))/16 + (15*dq3*dqr2*cos(2*q4)*sin(2*q5))/64 + (3*dq3*dqr2*cos(2*q5)*sin(2*q4))/16 - (15*dq3*dqr3*cos(2*q4)*sin(2*q5))/64 - (3*dq3*dqr3*cos(2*q5)*sin(2*q4))/16 + (3^(1/2)*ddqr2*cos(q4)*cos(q5))/8 - (3^(1/2)*ddqr3*cos(q4)*cos(q5))/8 - (3*dq1*dqr3*cos(q2)*sin(q3))/16 + (3*dq1*dqr3*cos(q3)*sin(q2))/16 - (3^(1/2)*ddqr2*sin(q4)*sin(q5))/4 + (3^(1/2)*ddqr3*sin(q4)*sin(q5))/4 - (9*dq1*dqr4*sin(2*q5)*cos(q2)*cos(q3))/32 - (9*dq1*dqr4*sin(2*q5)*sin(q2)*sin(q3))/32 - (3*3^(1/2)*dq2*dqr4*cos(q4)*sin(q5))/16 - (3*3^(1/2)*dq4*dqr2*cos(q4)*sin(q5))/16 + (3*3^(1/2)*dq3*dqr4*cos(q4)*sin(q5))/16 + (3*3^(1/2)*dq4*dqr3*cos(q4)*sin(q5))/16 + (3*3^(1/2)*dq2*dqr4*cos(2*q5)*sin(q4))/16 + (3*3^(1/2)*dq2*dqr4*sin(2*q5)*cos(q4))/32 + (3*3^(1/2)*dq4*dqr2*cos(2*q5)*sin(q4))/16 + (3*3^(1/2)*dq4*dqr2*sin(2*q5)*cos(q4))/32 - (3*3^(1/2)*dq3*dqr4*cos(2*q5)*sin(q4))/16 - (3*3^(1/2)*dq3*dqr4*sin(2*q5)*cos(q4))/32 - (3*3^(1/2)*dq4*dqr3*cos(2*q5)*sin(q4))/16 - (3*3^(1/2)*dq4*dqr3*sin(2*q5)*cos(q4))/32 + (3*dq1*dqr3*cos(q2)*cos(q5)*sin(q3))/16 - (3*dq1*dqr3*cos(q3)*cos(q5)*sin(q2))/16 - (3*dq1*dqr4*cos(q2)*cos(q3)*sin(q5))/16 - (3*3^(1/2)*ddqr1*cos(q2)*sin(q3)*sin(q4))/8 + (3*3^(1/2)*ddqr1*cos(q3)*sin(q2)*sin(q4))/8 - (3*dq1*dqr4*sin(q2)*sin(q3)*sin(q5))/16 + (3*dq1*dqr3*sin(2*q4)*cos(q2)*sin(q3)*sin(q5))/32 - (3*dq1*dqr3*sin(2*q4)*cos(q3)*sin(q2)*sin(q5))/32 + (3*3^(1/2)*dq1*dqr2*cos(q2)*cos(q3)*sin(q4))/16 - (3*3^(1/2)*dq1*dqr3*cos(q2)*cos(q3)*sin(q4))/16 - (3*3^(1/2)*dq1*dqr4*cos(q2)*cos(q4)*sin(q3))/16 + (3*3^(1/2)*dq1*dqr4*cos(q3)*cos(q4)*sin(q2))/16 - (3*3^(1/2)*dq1*dqr3*sin(q2)*sin(q3)*sin(q4))/16 + (3*dq1*dqr3*cos(2*q4)*cos(2*q5)*cos(q2)*sin(q3))/16 - (3*dq1*dqr3*cos(2*q4)*cos(2*q5)*cos(q3)*sin(q2))/16 - (15*dq1*dqr3*sin(2*q4)*sin(2*q5)*cos(q2)*sin(q3))/64 + (15*dq1*dqr3*sin(2*q4)*sin(2*q5)*cos(q3)*sin(q2))/64 - (3^(1/2)*ddqr1*cos(q2)*cos(q4)*sin(q3)*sin(q5))/4 - (3^(1/2)*ddqr1*cos(q2)*cos(q5)*sin(q3)*sin(q4))/8 + (3^(1/2)*ddqr1*cos(q3)*cos(q4)*sin(q2)*sin(q5))/4 + (3^(1/2)*ddqr1*cos(q3)*cos(q5)*sin(q2)*sin(q4))/8 - (3*dq1*dqr3*cos(2*q4)*cos(q2)*cos(q5)*sin(q3))/16 + (3*dq1*dqr3*cos(2*q4)*cos(q3)*cos(q5)*sin(q2))/16 - (3^(1/2)*dq1*dqr3*cos(q4)*sin(q2)*sin(q3)*sin(q5))/16 - (3^(1/2)*dq1*dqr3*cos(q5)*sin(q2)*sin(q3)*sin(q4))/8 + (3*3^(1/2)*dq1*dqr4*cos(q2)*sin(q3)*sin(q4)*sin(q5))/16 - (3*3^(1/2)*dq1*dqr4*cos(q3)*sin(q2)*sin(q4)*sin(q5))/16 + (3*3^(1/2)*dq1*dqr2*cos(2*q5)*cos(q2)*cos(q3)*sin(q4))/16 + (3*3^(1/2)*dq1*dqr2*sin(2*q5)*cos(q2)*cos(q3)*cos(q4))/32 - (3*3^(1/2)*dq1*dqr3*cos(2*q5)*cos(q2)*cos(q3)*sin(q4))/16 - (3*3^(1/2)*dq1*dqr3*sin(2*q5)*cos(q2)*cos(q3)*cos(q4))/32 + (3*3^(1/2)*dq1*dqr4*cos(2*q5)*cos(q2)*cos(q4)*sin(q3))/16 - (3*3^(1/2)*dq1*dqr4*cos(2*q5)*cos(q3)*cos(q4)*sin(q2))/16 - (3*3^(1/2)*dq1*dqr3*cos(2*q5)*sin(q2)*sin(q3)*sin(q4))/16 - (3*3^(1/2)*dq1*dqr3*sin(2*q5)*cos(q4)*sin(q2)*sin(q3))/32 - (3*3^(1/2)*dq1*dqr4*sin(2*q5)*cos(q2)*sin(q3)*sin(q4))/32 + (3*3^(1/2)*dq1*dqr4*sin(2*q5)*cos(q3)*sin(q2)*sin(q4))/32 + (3^(1/2)*dq1*dqr2*cos(q2)*cos(q3)*cos(q4)*sin(q5))/16 - (3^(1/2)*dq1*dqr3*cos(q2)*cos(q3)*cos(q4)*sin(q5))/16 - (3^(1/2)*dq1*dqr3*cos(q2)*cos(q3)*cos(q5)*sin(q4))/8;
Y5_24_1=(3*sin(q2)*sin(q3)*sin(q5))/4 + (3*cos(q2)*cos(q3)*sin(q5))/4 - (3^(1/2)*cos(q2)*cos(q4)*cos(q5)*sin(q3))/2 + (3^(1/2)*cos(q3)*cos(q4)*cos(q5)*sin(q2))/2 + (3^(1/2)*cos(q2)*sin(q3)*sin(q4)*sin(q5))/4 - (3^(1/2)*cos(q3)*sin(q2)*sin(q4)*sin(q5))/4;
Y1_1=Y1_1_1; 
Y1_2=Y1_2_1; 
Y1_3=Y1_3_1; 
Y1_4=Y1_4_1 + Y1_4_2; 
Y1_5=Y1_5_1 + Y1_5_2 + Y1_5_3 + Y1_5_4 + Y1_5_5 + Y1_5_6 + Y1_5_7 + Y1_5_8; 
Y1_6=Y1_6_1; 
Y1_7=Y1_7_1; 
Y1_8=Y1_8_1; 
Y1_9=Y1_9_1 + Y1_9_2; 
Y1_10=Y1_10_1 + Y1_10_2 + Y1_10_3 + Y1_10_4 + Y1_10_5 + Y1_10_6 + Y1_10_7 + Y1_10_8; 
Y1_15=Y1_15_1; 
Y1_16=Y1_16_1; 
Y1_17=Y1_17_1; 
Y1_18=Y1_18_1; 
Y1_19=Y1_19_1 + Y1_19_2 + Y1_19_3 + Y1_19_4 + Y1_19_5 + Y1_19_6; 
Y2_2=Y2_2_1; 
Y2_3=Y2_3_1; 
Y2_4=Y2_4_1; 
Y2_5=Y2_5_1 + Y2_5_2 + Y2_5_3 + Y2_5_4; 
Y2_6=Y2_6_1; 
Y2_7=Y2_7_1; 
Y2_8=Y2_8_1; 
Y2_9=Y2_9_1; 
Y2_10=Y2_10_1 + Y2_10_2 + Y2_10_3 + Y2_10_4; 
Y2_11=Y2_11_1; 
Y2_12=Y2_12_1; 
Y2_13=Y2_13_1; 
Y2_14=Y2_14_1; 
Y2_15=Y2_15_1; 
Y2_16=Y2_16_1; 
Y2_17=Y2_17_1; 
Y2_18=Y2_18_1; 
Y2_19=Y2_19_1 + Y2_19_2 + Y2_19_3; 
Y2_20=Y2_20_1; 
Y2_21=Y2_21_1; 
Y2_22=Y2_22_1; 
Y2_23=Y2_23_1; 
Y2_24=Y2_24_1; 
Y3_3=Y3_3_1; 
Y3_4=Y3_4_1; 
Y3_5=Y3_5_1 + Y3_5_2 + Y3_5_3; 
Y3_7=Y3_7_1; 
Y3_8=Y3_8_1; 
Y3_9=Y3_9_1; 
Y3_10=Y3_10_1 + Y3_10_2 + Y3_10_3; 
Y3_12=Y3_12_1; 
Y3_13=Y3_13_1; 
Y3_14=Y3_14_1; 
Y3_16=Y3_16_1; 
Y3_17=Y3_17_1; 
Y3_18=Y3_18_1; 
Y3_19=Y3_19_1 + Y3_19_2 + Y3_19_3; 
Y3_21=Y3_21_1; 
Y3_22=Y3_22_1; 
Y3_23=Y3_23_1; 
Y3_24=Y3_24_1; 
Y4_4=Y4_4_1; 
Y4_5=Y4_5_1 + Y4_5_2 + Y4_5_3; 
Y4_9=Y4_9_1; 
Y4_10=Y4_10_1 + Y4_10_2 + Y4_10_3; 
Y4_13=Y4_13_1; 
Y4_14=Y4_14_1; 
Y4_18=Y4_18_1; 
Y4_19=Y4_19_1 + Y4_19_2 + Y4_19_3; 
Y4_23=Y4_23_1; 
Y4_24=Y4_24_1; 
Y5_5=Y5_5_1 + Y5_5_2 + Y5_5_3; 
Y5_10=Y5_10_1 + Y5_10_2 + Y5_10_3; 
Y5_14=Y5_14_1; 
Y5_19=Y5_19_1 + Y5_19_2; 
Y5_24=Y5_24_1; 
Y=[Y1_1, Y1_2, Y1_3, Y1_4, Y1_5, Y1_6, Y1_7, Y1_8, Y1_9, Y1_10, 0, 0, 0, 0, Y1_15, Y1_16, Y1_17, Y1_18, Y1_19, 0, 0, 0, 0, 0;
0, Y2_2, Y2_3, Y2_4, Y2_5, Y2_6, Y2_7, Y2_8, Y2_9, Y2_10, Y2_11, Y2_12, Y2_13, Y2_14, Y2_15, Y2_16, Y2_17, Y2_18, Y2_19, Y2_20, Y2_21, Y2_22, Y2_23, Y2_24;
0, 0, Y3_3, Y3_4, Y3_5, 0, Y3_7, Y3_8, Y3_9, Y3_10, 0, Y3_12, Y3_13, Y3_14, 0, Y3_16, Y3_17, Y3_18, Y3_19, 0, Y3_21, Y3_22, Y3_23, Y3_24;
0, 0, 0, Y4_4, Y4_5, 0, 0, 0, Y4_9, Y4_10, 0, 0, Y4_13, Y4_14, 0, 0, 0, Y4_18, Y4_19, 0, 0, 0, Y4_23, Y4_24;
0, 0, 0, 0, Y5_5, 0, 0, 0, 0, Y5_10, 0, 0, 0, Y5_14, 0, 0, 0, 0, Y5_19, 0, 0, 0, 0, Y5_24;
0, 0, 0, 0, 0, 0, 0, 0, 0, 0, 0, 0, 0, 0, 0, 0, 0, 0, 0, 0, 0, 0, 0, 0];
